simulink model "ForwardKinematic_YuMi"  (R2024a)
(part 22 of 23)

(4503599440548691*sin(q4R))/4503599627370496)*((7514214926474921*sin(q3R)*((4774755754024928798560446539205*cos(q2R))/10141204801825835211973625643008 + (7514214926474921*cos(q2R)*((3148506117433717*cos(q1R))/4503599627370496 + (1211728953682539*sin(q1R))/2251799813685248))/36893488147419103232 - sin(q2R)*((1211728953682539*cos(q1R))/2251799813685248 - (3148506117433717*sin(q1R))/4503599627370496)))/36893488147419103232 - cos(q3R)*((4774755754024928798560446539205*sin(q2R))/10141204801825835211973625643008 + cos(q2R)*((1211728953682539*cos(q1R))/2251799813685248 - (3148506117433717*sin(q1R))/4503599627370496) + (7514214926474921*sin(q2R)*((3148506117433717*cos(q1R))/4503599627370496 + (1211728953682539*sin(q1R))/2251799813685248))/36893488147419103232) + (9007199067919185*sin(q3R)*((28359221366286827792295350160645*cos(q1R))/40564819207303340847894502572032 + (10914283902180054573281797610715*sin(q1R))/20282409603651670423947251286016 - 3983318308679801924058395430653/41538374868278621028243970633760768))/9007199254740992) - ((9007199067919185*cos(q4R))/9007199254740992 - (234819211581865*sin(q4R))/1152921504606846976)*((213097284493758984364555654519459856780913684045*cos(q1R))/1496577676626844588240573268701473812127674924007424 - (43007175577195104036898489188735438973874147925*cos(q2R))/91343852333181432387730302044767688728495783936 + (82012275009546312639155898108543355135168378515*sin(q1R))/748288838313422294120286634350736906063837462003712 - (67682029681889335677290557259385*cos(q2R)*((3148506117433717*cos(q1R))/4503599627370496 + (1211728953682539*sin(q1R))/2251799813685248))/332306998946228968225951765070086144 + (9007199067919185*sin(q2R)*((1211728953682539*cos(q1R))/2251799813685248 - (3148506117433717*sin(q1R))/4503599627370496))/9007199254740992 - 29931509891982604486959633650198707742999153413/1532495540865888858358347027150309183618739122183602176) + (7514214926474921*sin(q4R)*((7514214926474921*cos(q3R)*((4774755754024928798560446539205*cos(q2R))/10141204801825835211973625643008 + (7514214926474921*cos(q2R)*((3148506117433717*cos(q1R))/4503599627370496 + (1211728953682539*sin(q1R))/2251799813685248))/36893488147419103232 - sin(q2R)*((1211728953682539*cos(q1R))/2251799813685248 - (3148506117433717*sin(q1R))/4503599627370496)))/36893488147419103232 + sin(q3R)*((4774755754024928798560446539205*sin(q2R))/10141204801825835211973625643008 + cos(q2R)*((1211728953682539*cos(q1R))/2251799813685248 - (3148506117433717*sin(q1R))/4503599627370496) + (7514214926474921*sin(q2R)*((3148506117433717*cos(q1R))/4503599627370496 + (1211728953682539*sin(q1R))/2251799813685248))/36893488147419103232) + (9007199067919185*cos(q3R)*((28359221366286827792295350160645*cos(q1R))/40564819207303340847894502572032 + (10914283902180054573281797610715*sin(q1R))/20282409603651670423947251286016 - 3983318308679801924058395430653/41538374868278621028243970633760768))/9007199254740992))/36893488147419103232))/36893488147419103232 + cos(q5R)*(((4503599440548691*cos(q4R))/4503599627370496 - (7514214926474921*sin(q4R))/36893488147419103232)*((7514214926474921*sin(q3R)*((4774755754024928798560446539205*cos(q2R))/10141204801825835211973625643008 + (7514214926474921*cos(q2R)*((3148506117433717*cos(q1R))/4503599627370496 + (1211728953682539*sin(q1R))/2251799813685248))/36893488147419103232 - sin(q2R)*((1211728953682539*cos(q1R))/2251799813685248 - (3148506117433717*sin(q1R))/4503599627370496)))/36893488147419103232 - cos(q3R)*((4774755754024928798560446539205*sin(q2R))/10141204801825835211973625643008 + cos(q2R)*((1211728953682539*cos(q1R))/2251799813685248 - (3148506117433717*sin(q1R))/4503599627370496) + (7514214926474921*sin(q2R)*((3148506117433717*cos(q1R))/4503599627370496 + (1211728953682539*sin(q1R))/2251799813685248))/36893488147419103232) + (9007199067919185*sin(q3R)*((28359221366286827792295350160645*cos(q1R))/40564819207303340847894502572032 + (10914283902180054573281797610715*sin(q1R))/20282409603651670423947251286016 - 3983318308679801924058395430653/41538374868278621028243970633760768))/9007199254740992) + ((234819211581865*cos(q4R))/1152921504606846976 + (9007199067919185*sin(q4R))/9007199254740992)*((213097284493758984364555654519459856780913684045*cos(q1R))/1496577676626844588240573268701473812127674924007424 - (43007175577195104036898489188735438973874147925*cos(q2R))/91343852333181432387730302044767688728495783936 + (82012275009546312639155898108543355135168378515*sin(q1R))/748288838313422294120286634350736906063837462003712 - (67682029681889335677290557259385*cos(q2R)*((3148506117433717*cos(q1R))/4503599627370496 + (1211728953682539*sin(q1R))/2251799813685248))/332306998946228968225951765070086144 + (9007199067919185*sin(q2R)*((1211728953682539*cos(q1R))/2251799813685248 - (3148506117433717*sin(q1R))/4503599627370496))/9007199254740992 - 29931509891982604486959633650198707742999153413/1532495540865888858358347027150309183618739122183602176) + (7514214926474921*cos(q4R)*((7514214926474921*cos(q3R)*((4774755754024928798560446539205*cos(q2R))/10141204801825835211973625643008 + (7514214926474921*cos(q2R)*((3148506117433717*cos(q1R))/4503599627370496 + (1211728953682539*sin(q1R))/2251799813685248))/36893488147419103232 - sin(q2R)*((1211728953682539*cos(q1R))/2251799813685248 - (3148506117433717*sin(q1R))/4503599627370496)))/36893488147419103232 + sin(q3R)*((4774755754024928798560446539205*sin(q2R))/10141204801825835211973625643008 + cos(q2R)*((1211728953682539*cos(q1R))/2251799813685248 - (3148506117433717*sin(q1R))/4503599627370496) + (7514214926474921*sin(q2R)*((3148506117433717*cos(q1R))/4503599627370496 + (1211728953682539*sin(q1R))/2251799813685248))/36893488147419103232) + (9007199067919185*cos(q3R)*((28359221366286827792295350160645*cos(q1R))/40564819207303340847894502572032 + (10914283902180054573281797610715*sin(q1R))/20282409603651670423947251286016 - 3983318308679801924058395430653/41538374868278621028243970633760768))/9007199254740992))/36893488147419103232)))/9007199254740992000 + (81*((4503599440548691*cos(q4R))/4503599627370496 - (7514214926474921*sin(q4R))/36893488147419103232)*((7514214926474921*sin(q3R)*((4774755754024928798560446539205*cos(q2R))/10141204801825835211973625643008 + (7514214926474921*cos(q2R)*((3148506117433717*cos(q1R))/4503599627370496 + (1211728953682539*sin(q1R))/2251799813685248))/36893488147419103232 - sin(q2R)*((1211728953682539*cos(q1R))/2251799813685248 - (3148506117433717*sin(q1R))/4503599627370496)))/36893488147419103232 - cos(q3R)*((4774755754024928798560446539205*sin(q2R))/10141204801825835211973625643008 + cos(q2R)*((1211728953682539*cos(q1R))/2251799813685248 - (3148506117433717*sin(q1R))/4503599627370496) + (7514214926474921*sin(q2R)*((3148506117433717*cos(q1R))/4503599627370496 + (1211728953682539*sin(q1R))/2251799813685248))/36893488147419103232) + (9007199067919185*sin(q3R)*((28359221366286827792295350160645*cos(q1R))/40564819207303340847894502572032 + (10914283902180054573281797610715*sin(q1R))/20282409603651670423947251286016 - 3983318308679801924058395430653/41538374868278621028243970633760768))/9007199254740992))/2000 - (81222263116692158804177042061221826384594597321566869716687*((7514214926474921*cos(q4R))/36893488147419103232 + (4503599440548691*sin(q4R))/4503599627370496)*((7514214926474921*sin(q3R)*((4774755754024928798560446539205*cos(q2R))/10141204801825835211973625643008 + (7514214926474921*cos(q2R)*((3148506117433717*cos(q1R))/4503599627370496 + (1211728953682539*sin(q1R))/2251799813685248))/36893488147419103232 - sin(q2R)*((1211728953682539*cos(q1R))/2251799813685248 - (3148506117433717*sin(q1R))/4503599627370496)))/36893488147419103232 - cos(q3R)*((4774755754024928798560446539205*sin(q2R))/10141204801825835211973625643008 + cos(q2R)*((1211728953682539*cos(q1R))/2251799813685248 - (3148506117433717*sin(q1R))/4503599627370496) + (7514214926474921*sin(q2R)*((3148506117433717*cos(q1R))/4503599627370496 + (1211728953682539*sin(q1R))/2251799813685248))/36893488147419103232) + (9007199067919185*sin(q3R)*((28359221366286827792295350160645*cos(q1R))/40564819207303340847894502572032 + (10914283902180054573281797610715*sin(q1R))/20282409603651670423947251286016 - 3983318308679801924058395430653/41538374868278621028243970633760768))/9007199254740992))/306499108173177771671669405430061836723747824436720435200000 + (81222263116692158804177042061221826384594597321566869716687*((9007199067919185*cos(q4R))/9007199254740992 - (234819211581865*sin(q4R))/1152921504606846976)*((213097284493758984364555654519459856780913684045*cos(q1R))/1496577676626844588240573268701473812127674924007424 - (43007175577195104036898489188735438973874147925*cos(q2R))/91343852333181432387730302044767688728495783936 + (82012275009546312639155898108543355135168378515*sin(q1R))/748288838313422294120286634350736906063837462003712 - (67682029681889335677290557259385*cos(q2R)*((3148506117433717*cos(q1R))/4503599627370496 + (1211728953682539*sin(q1R))/2251799813685248))/332306998946228968225951765070086144 + (9007199067919185*sin(q2R)*((1211728953682539*cos(q1R))/2251799813685248 - (3148506117433717*sin(q1R))/4503599627370496))/9007199254740992 - 29931509891982604486959633650198707742999153413/1532495540865888858358347027150309183618739122183602176))/306499108173177771671669405430061836723747824436720435200000 + (81*((234819211581865*cos(q4R))/1152921504606846976 + (9007199067919185*sin(q4R))/9007199254740992)*((213097284493758984364555654519459856780913684045*cos(q1R))/1496577676626844588240573268701473812127674924007424 - (43007175577195104036898489188735438973874147925*cos(q2R))/91343852333181432387730302044767688728495783936 + (82012275009546312639155898108543355135168378515*sin(q1R))/748288838313422294120286634350736906063837462003712 - (67682029681889335677290557259385*cos(q2R)*((3148506117433717*cos(q1R))/4503599627370496 + (1211728953682539*sin(q1R))/2251799813685248))/332306998946228968225951765070086144 + (9007199067919185*sin(q2R)*((1211728953682539*cos(q1R))/2251799813685248 - (3148506117433717*sin(q1R))/4503599627370496))/9007199254740992 - 29931509891982604486959633650198707742999153413/1532495540865888858358347027150309183618739122183602176))/2000 - (584133382113593486367040631332731*cos(q6R)*((9007199067919185*((7514214926474921*cos(q4R))/36893488147419103232 + (4503599440548691*sin(q4R))/4503599627370496)*((7514214926474921*sin(q3R)*((4774755754024928798560446539205*cos(q2R))/10141204801825835211973625643008 + (7514214926474921*cos(q2R)*((3148506117433717*cos(q1R))/4503599627370496 + (1211728953682539*sin(q1R))/2251799813685248))/36893488147419103232 - sin(q2R)*((1211728953682539*cos(q1R))/2251799813685248 - (3148506117433717*sin(q1R))/4503599627370496)))/36893488147419103232 - cos(q3R)*((4774755754024928798560446539205*sin(q2R))/10141204801825835211973625643008 + cos(q2R)*((1211728953682539*cos(q1R))/2251799813685248 - (3148506117433717*sin(q1R))/4503599627370496) + (7514214926474921*sin(q2R)*((3148506117433717*cos(q1R))/4503599627370496 + (1211728953682539*sin(q1R))/2251799813685248))/36893488147419103232) + (9007199067919185*sin(q3R)*((28359221366286827792295350160645*cos(q1R))/40564819207303340847894502572032 + (10914283902180054573281797610715*sin(q1R))/20282409603651670423947251286016 - 3983318308679801924058395430653/41538374868278621028243970633760768))/9007199254740992))/9007199254740992 - (9007199067919185*((9007199067919185*cos(q4R))/9007199254740992 - (234819211581865*sin(q4R))/1152921504606846976)*((213097284493758984364555654519459856780913684045*cos(q1R))/1496577676626844588240573268701473812127674924007424 - (43007175577195104036898489188735438973874147925*cos(q2R))/91343852333181432387730302044767688728495783936 + (82012275009546312639155898108543355135168378515*sin(q1R))/748288838313422294120286634350736906063837462003712 - (67682029681889335677290557259385*cos(q2R)*((3148506117433717*cos(q1R))/4503599627370496 + (1211728953682539*sin(q1R))/2251799813685248))/332306998946228968225951765070086144 + (9007199067919185*sin(q2R)*((1211728953682539*cos(q1R))/2251799813685248 - (3148506117433717*sin(q1R))/4503599627370496))/9007199254740992 - 29931509891982604486959633650198707742999153413/1532495540865888858358347027150309183618739122183602176))/9007199254740992 + (67682029681889335677290557259385*sin(q4R)*((7514214926474921*cos(q3R)*((4774755754024928798560446539205*cos(q2R))/10141204801825835211973625643008 + (7514214926474921*cos(q2R)*((3148506117433717*cos(q1R))/4503599627370496 + (1211728953682539*sin(q1R))/2251799813685248))/36893488147419103232 - sin(q2R)*((1211728953682539*cos(q1R))/2251799813685248 - (3148506117433717*sin(q1R))/4503599627370496)))/36893488147419103232 + sin(q3R)*((4774755754024928798560446539205*sin(q2R))/10141204801825835211973625643008 + cos(q2R)*((1211728953682539*cos(q1R))/2251799813685248 - (3148506117433717*sin(q1R))/4503599627370496) + (7514214926474921*sin(q2R)*((3148506117433717*cos(q1R))/4503599627370496 + (1211728953682539*sin(q1R))/2251799813685248))/36893488147419103232) + (9007199067919185*cos(q3R)*((28359221366286827792295350160645*cos(q1R))/40564819207303340847894502572032 + (10914283902180054573281797610715*sin(q1R))/20282409603651670423947251286016 - 3983318308679801924058395430653/41538374868278621028243970633760768))/9007199254740992))/332306998946228968225951765070086144))/16225927682921336339157801028812800 - (48638874966763599*sin(q6R)*((9007199067919185*((7514214926474921*cos(q4R))/36893488147419103232 + (4503599440548691*sin(q4R))/4503599627370496)*((7514214926474921*sin(q3R)*((4774755754024928798560446539205*cos(q2R))/10141204801825835211973625643008 + (7514214926474921*cos(q2R)*((3148506117433717*cos(q1R))/4503599627370496 + (1211728953682539*sin(q1R))/2251799813685248))/36893488147419103232 - sin(q2R)*((1211728953682539*cos(q1R))/2251799813685248 - (3148506117433717*sin(q1R))/4503599627370496)))/36893488147419103232 - cos(q3R)*((4774755754024928798560446539205*sin(q2R))/10141204801825835211973625643008 + cos(q2R)*((1211728953682539*cos(q1R))/2251799813685248 - (3148506117433717*sin(q1R))/4503599627370496) + (7514214926474921*sin(q2R)*((3148506117433717*cos(q1R))/4503599627370496 + (1211728953682539*sin(q1R))/2251799813685248))/36893488147419103232) + (9007199067919185*sin(q3R)*((28359221366286827792295350160645*cos(q1R))/40564819207303340847894502572032 + (10914283902180054573281797610715*sin(q1R))/20282409603651670423947251286016 - 3983318308679801924058395430653/41538374868278621028243970633760768))/9007199254740992))/9007199254740992 - (9007199067919185*((9007199067919185*cos(q4R))/9007199254740992 - (234819211581865*sin(q4R))/1152921504606846976)*((213097284493758984364555654519459856780913684045*cos(q1R))/1496577676626844588240573268701473812127674924007424 - (43007175577195104036898489188735438973874147925*cos(q2R))/91343852333181432387730302044767688728495783936 + (82012275009546312639155898108543355135168378515*sin(q1R))/748288838313422294120286634350736906063837462003712 - (67682029681889335677290557259385*cos(q2R)*((3148506117433717*cos(q1R))/4503599627370496 + (1211728953682539*sin(q1R))/2251799813685248))/332306998946228968225951765070086144 + (9007199067919185*sin(q2R)*((1211728953682539*cos(q1R))/2251799813685248 - (3148506117433717*sin(q1R))/4503599627370496))/9007199254740992 - 29931509891982604486959633650198707742999153413/1532495540865888858358347027150309183618739122183602176))/9007199254740992 + (67682029681889335677290557259385*sin(q4R)*((7514214926474921*cos(q3R)*((4774755754024928798560446539205*cos(q2R))/10141204801825835211973625643008 + (7514214926474921*cos(q2R)*((3148506117433717*cos(q1R))/4503599627370496 + (1211728953682539*sin(q1R))/2251799813685248))/36893488147419103232 - sin(q2R)*((1211728953682539*cos(q1R))/2251799813685248 - (3148506117433717*sin(q1R))/4503599627370496)))/36893488147419103232 + sin(q3R)*((4774755754024928798560446539205*sin(q2R))/10141204801825835211973625643008 + cos(q2R)*((1211728953682539*cos(q1R))/2251799813685248 - (3148506117433717*sin(q1R))/4503599627370496) + (7514214926474921*sin(q2R)*((3148506117433717*cos(q1R))/4503599627370496 + (1211728953682539*sin(q1R))/2251799813685248))/36893488147419103232) + (9007199067919185*cos(q3R)*((28359221366286827792295350160645*cos(q1R))/40564819207303340847894502572032 + (10914283902180054573281797610715*sin(q1R))/20282409603651670423947251286016 - 3983318308679801924058395430653/41538374868278621028243970633760768))/9007199254740992))/332306998946228968225951765070086144))/1801439850948198400 + (608651409044468601*cos(q4R)*((7514214926474921*cos(q3R)*((4774755754024928798560446539205*cos(q2R))/10141204801825835211973625643008 + (7514214926474921*cos(q2R)*((3148506117433717*cos(q1R))/4503599627370496 + (1211728953682539*sin(q1R))/2251799813685248))/36893488147419103232 - sin(q2R)*((1211728953682539*cos(q1R))/2251799813685248 - (3148506117433717*sin(q1R))/4503599627370496)))/36893488147419103232 + sin(q3R)*((4774755754024928798560446539205*sin(q2R))/10141204801825835211973625643008 + cos(q2R)*((1211728953682539*cos(q1R))/2251799813685248 - (3148506117433717*sin(q1R))/4503599627370496) + (7514214926474921*sin(q2R)*((3148506117433717*cos(q1R))/4503599627370496 + (1211728953682539*sin(q1R))/2251799813685248))/36893488147419103232) + (9007199067919185*cos(q3R)*((28359221366286827792295350160645*cos(q1R))/40564819207303340847894502572032 + (10914283902180054573281797610715*sin(q1R))/20282409603651670423947251286016 - 3983318308679801924058395430653/41538374868278621028243970633760768))/9007199254740992))/73786976294838206464000 - (27*cos(q5R)*(((4503599440548691*cos(q4R))/4503599627370496 - (7514214926474921*sin(q4R))/36893488147419103232)*((7514214926474921*sin(q3R)*((4774755754024928798560446539205*cos(q2R))/10141204801825835211973625643008 + (7514214926474921*cos(q2R)*((3148506117433717*cos(q1R))/4503599627370496 + (1211728953682539*sin(q1R))/2251799813685248))/36893488147419103232 - sin(q2R)*((1211728953682539*cos(q1R))/2251799813685248 - (3148506117433717*sin(q1R))/4503599627370496)))/36893488147419103232 - cos(q3R)*((4774755754024928798560446539205*sin(q2R))/10141204801825835211973625643008 + cos(q2R)*((1211728953682539*cos(q1R))/2251799813685248 - (3148506117433717*sin(q1R))/4503599627370496) + (7514214926474921*sin(q2R)*((3148506117433717*cos(q1R))/4503599627370496 + (1211728953682539*sin(q1R))/2251799813685248))/36893488147419103232) + (9007199067919185*sin(q3R)*((28359221366286827792295350160645*cos(q1R))/40564819207303340847894502572032 + (10914283902180054573281797610715*sin(q1R))/20282409603651670423947251286016 - 3983318308679801924058395430653/41538374868278621028243970633760768))/9007199254740992) + ((234819211581865*cos(q4R))/1152921504606846976 + (9007199067919185*sin(q4R))/9007199254740992)*((213097284493758984364555654519459856780913684045*cos(q1R))/1496577676626844588240573268701473812127674924007424 - (43007175577195104036898489188735438973874147925*cos(q2R))/91343852333181432387730302044767688728495783936 + (82012275009546312639155898108543355135168378515*sin(q1R))/748288838313422294120286634350736906063837462003712 - (67682029681889335677290557259385*cos(q2R)*((3148506117433717*cos(q1R))/4503599627370496 + (1211728953682539*sin(q1R))/2251799813685248))/332306998946228968225951765070086144 + (9007199067919185*sin(q2R)*((1211728953682539*cos(q1R))/2251799813685248 - (3148506117433717*sin(q1R))/4503599627370496))/9007199254740992 - 29931509891982604486959633650198707742999153413/1532495540865888858358347027150309183618739122183602176) + (7514214926474921*cos(q4R)*((7514214926474921*cos(q3R)*((4774755754024928798560446539205*cos(q2R))/10141204801825835211973625643008 + (7514214926474921*cos(q2R)*((3148506117433717*cos(q1R))/4503599627370496 + (1211728953682539*sin(q1R))/2251799813685248))/36893488147419103232 - sin(q2R)*((1211728953682539*cos(q1R))/2251799813685248 - (3148506117433717*sin(q1R))/4503599627370496)))/36893488147419103232 + sin(q3R)*((4774755754024928798560446539205*sin(q2R))/10141204801825835211973625643008 + cos(q2R)*((1211728953682539*cos(q1R))/2251799813685248 - (3148506117433717*sin(q1R))/4503599627370496) + (7514214926474921*sin(q2R)*((3148506117433717*cos(q1R))/4503599627370496 + (1211728953682539*sin(q1R))/2251799813685248))/36893488147419103232) + (9007199067919185*cos(q3R)*((28359221366286827792295350160645*cos(q1R))/40564819207303340847894502572032 + (10914283902180054573281797610715*sin(q1R))/20282409603651670423947251286016 - 3983318308679801924058395430653/41538374868278621028243970633760768))/9007199254740992))/36893488147419103232))/1000 - (610321541873521657855151997354401418608858870661075444886782706002880706727*sin(q4R)*((7514214926474921*cos(q3R)*((4774755754024928798560446539205*cos(q2R))/10141204801825835211973625643008 + (7514214926474921*cos(q2R)*((3148506117433717*cos(q1R))/4503599627370496 + (1211728953682539*sin(q1R))/2251799813685248))/36893488147419103232 - sin(q2R)*((1211728953682539*cos(q1R))/2251799813685248 - (3148506117433717*sin(q1R))/4503599627370496)))/36893488147419103232 + sin(q3R)*((4774755754024928798560446539205*sin(q2R))/10141204801825835211973625643008 + cos(q2R)*((1211728953682539*cos(q1R))/2251799813685248 - (3148506117433717*sin(q1R))/4503599627370496) + (7514214926474921*sin(q2R)*((3148506117433717*cos(q1R))/4503599627370496 + (1211728953682539*sin(q1R))/2251799813685248))/36893488147419103232) + (9007199067919185*cos(q3R)*((28359221366286827792295350160645*cos(q1R))/40564819207303340847894502572032 + (10914283902180054573281797610715*sin(q1R))/20282409603651670423947251286016 - 3983318308679801924058395430653/41538374868278621028243970633760768))/9007199254740992))/11307821214581659709333104004754678501295896940003961331978279688272766566400000 - (94754841554645069948206780163139*sin(q5R)*(((4503599440548691*cos(q4R))/4503599627370496 - (7514214926474921*sin(q4R))/36893488147419103232)*((7514214926474921*sin(q3R)*((4774755754024928798560446539205*cos(q2R))/10141204801825835211973625643008 + (7514214926474921*cos(q2R)*((3148506117433717*cos(q1R))/4503599627370496 + (1211728953682539*sin(q1R))/2251799813685248))/36893488147419103232 - sin(q2R)*((1211728953682539*cos(q1R))/2251799813685248 - (3148506117433717*sin(q1R))/4503599627370496)))/36893488147419103232 - cos(q3R)*((4774755754024928798560446539205*sin(q2R))/10141204801825835211973625643008 + cos(q2R)*((1211728953682539*cos(q1R))/2251799813685248 - (3148506117433717*sin(q1R))/4503599627370496) + (7514214926474921*sin(q2R)*((3148506117433717*cos(q1R))/4503599627370496 + (1211728953682539*sin(q1R))/2251799813685248))/36893488147419103232) + (9007199067919185*sin(q3R)*((28359221366286827792295350160645*cos(q1R))/40564819207303340847894502572032 + (10914283902180054573281797610715*sin(q1R))/20282409603651670423947251286016 - 3983318308679801924058395430653/41538374868278621028243970633760768))/9007199254740992) + ((234819211581865*cos(q4R))/1152921504606846976 + (9007199067919185*sin(q4R))/9007199254740992)*((213097284493758984364555654519459856780913684045*cos(q1R))/1496577676626844588240573268701473812127674924007424 - (43007175577195104036898489188735438973874147925*cos(q2R))/91343852333181432387730302044767688728495783936 + (82012275009546312639155898108543355135168378515*sin(q1R))/748288838313422294120286634350736906063837462003712 - (67682029681889335677290557259385*cos(q2R)*((3148506117433717*cos(q1R))/4503599627370496 + (1211728953682539*sin(q1R))/2251799813685248))/332306998946228968225951765070086144 + (9007199067919185*sin(q2R)*((1211728953682539*cos(q1R))/2251799813685248 - (3148506117433717*sin(q1R))/4503599627370496))/9007199254740992 - 29931509891982604486959633650198707742999153413/1532495540865888858358347027150309183618739122183602176) + (7514214926474921*cos(q4R)*((7514214926474921*cos(q3R)*((4774755754024928798560446539205*cos(q2R))/10141204801825835211973625643008 + (7514214926474921*cos(q2R)*((3148506117433717*cos(q1R))/4503599627370496 + (1211728953682539*sin(q1R))/2251799813685248))/36893488147419103232 - sin(q2R)*((1211728953682539*cos(q1R))/2251799813685248 - (3148506117433717*sin(q1R))/4503599627370496)))/36893488147419103232 + sin(q3R)*((4774755754024928798560446539205*sin(q2R))/10141204801825835211973625643008 + cos(q2R)*((1211728953682539*cos(q1R))/2251799813685248 - (3148506117433717*sin(q1R))/4503599627370496) + (7514214926474921*sin(q2R)*((3148506117433717*cos(q1R))/4503599627370496 + (1211728953682539*sin(q1R))/2251799813685248))/36893488147419103232) + (9007199067919185*cos(q3R)*((28359221366286827792295350160645*cos(q1R))/40564819207303340847894502572032 + (10914283902180054573281797610715*sin(q1R))/20282409603651670423947251286016 - 3983318308679801924058395430653/41538374868278621028243970633760768))/9007199254740992))/36893488147419103232))/66461399789245793645190353014017228800 + (712008244765680093343103025701132101054572137019*cos(q5R)*(((7514214926474921*cos(q4R))/36893488147419103232 + (4503599440548691*sin(q4R))/4503599627370496)*((7514214926474921*sin(q3R)*((4774755754024928798560446539205*cos(q2R))/10141204801825835211973625643008 + (7514214926474921*cos(q2R)*((3148506117433717*cos(q1R))/4503599627370496 + (1211728953682539*sin(q1R))/2251799813685248))/36893488147419103232 - sin(q2R)*((1211728953682539*cos(q1R))/2251799813685248 - (3148506117433717*sin(q1R))/4503599627370496)))/36893488147419103232 - cos(q3R)*((4774755754024928798560446539205*sin(q2R))/10141204801825835211973625643008 + cos(q2R)*((1211728953682539*cos(q1R))/2251799813685248 - (3148506117433717*sin(q1R))/4503599627370496) + (7514214926474921*sin(q2R)*((3148506117433717*cos(q1R))/4503599627370496 + (1211728953682539*sin(q1R))/2251799813685248))/36893488147419103232) + (9007199067919185*sin(q3R)*((28359221366286827792295350160645*cos(q1R))/40564819207303340847894502572032 + (10914283902180054573281797610715*sin(q1R))/20282409603651670423947251286016 - 3983318308679801924058395430653/41538374868278621028243970633760768))/9007199254740992) - ((9007199067919185*cos(q4R))/9007199254740992 - (234819211581865*sin(q4R))/1152921504606846976)*((213097284493758984364555654519459856780913684045*cos(q1R))/1496577676626844588240573268701473812127674924007424 - (43007175577195104036898489188735438973874147925*cos(q2R))/91343852333181432387730302044767688728495783936 + (82012275009546312639155898108543355135168378515*sin(q1R))/748288838313422294120286634350736906063837462003712 - (67682029681889335677290557259385*cos(q2R)*((3148506117433717*cos(q1R))/4503599627370496 + (1211728953682539*sin(q1R))/2251799813685248))/332306998946228968225951765070086144 + (9007199067919185*sin(q2R)*((1211728953682539*cos(q1R))/2251799813685248 - (3148506117433717*sin(q1R))/4503599627370496))/9007199254740992 - 29931509891982604486959633650198707742999153413/1532495540865888858358347027150309183618739122183602176) + (7514214926474921*sin(q4R)*((7514214926474921*cos(q3R)*((4774755754024928798560446539205*cos(q2R))/10141204801825835211973625643008 + (7514214926474921*cos(q2R)*((3148506117433717*cos(q1R))/4503599627370496 + (1211728953682539*sin(q1R))/2251799813685248))/36893488147419103232 - sin(q2R)*((1211728953682539*cos(q1R))/2251799813685248 - (3148506117433717*sin(q1R))/4503599627370496)))/36893488147419103232 + sin(q3R)*((4774755754024928798560446539205*sin(q2R))/10141204801825835211973625643008 + cos(q2R)*((1211728953682539*cos(q1R))/2251799813685248 - (3148506117433717*sin(q1R))/4503599627370496) + (7514214926474921*sin(q2R)*((3148506117433717*cos(q1R))/4503599627370496 + (1211728953682539*sin(q1R))/2251799813685248))/36893488147419103232) + (9007199067919185*cos(q3R)*((28359221366286827792295350160645*cos(q1R))/40564819207303340847894502572032 + (10914283902180054573281797610715*sin(q1R))/20282409603651670423947251286016 - 3983318308679801924058395430653/41538374868278621028243970633760768))/9007199254740992))/36893488147419103232))/2451992865385422173373355243440494693789982595493763481600 + (2436553109258773196144549622003023*cos(q6R)*(sin(q5R)*(((4503599440548691*cos(q4R))/4503599627370496 - (7514214926474921*sin(q4R))/36893488147419103232)*((7514214926474921*sin(q3R)*((4774755754024928798560446539205*cos(q2R))/10141204801825835211973625643008 + (7514214926474921*cos(q2R)*((3148506117433717*cos(q1R))/4503599627370496 + (1211728953682539*sin(q1R))/2251799813685248))/36893488147419103232 - sin(q2R)*((1211728953682539*cos(q1R))/2251799813685248 - (3148506117433717*sin(q1R))/4503599627370496)))/36893488147419103232 - cos(q3R)*((4774755754024928798560446539205*sin(q2R))/10141204801825835211973625643008 + cos(q2R)*((1211728953682539*cos(q1R))/2251799813685248 - (3148506117433717*sin(q1R))/4503599627370496) + (7514214926474921*sin(q2R)*((3148506117433717*cos(q1R))/4503599627370496 + (1211728953682539*sin(q1R))/2251799813685248))/36893488147419103232) + (9007199067919185*sin(q3R)*((28359221366286827792295350160645*cos(q1R))/40564819207303340847894502572032 + (10914283902180054573281797610715*sin(q1R))/20282409603651670423947251286016 - 3983318308679801924058395430653/41538374868278621028243970633760768))/9007199254740992) + ((234819211581865*cos(q4R))/1152921504606846976 + (9007199067919185*sin(q4R))/9007199254740992)*((213097284493758984364555654519459856780913684045*cos(q1R))/1496577676626844588240573268701473812127674924007424 - (43007175577195104036898489188735438973874147925*cos(q2R))/91343852333181432387730302044767688728495783936 + (82012275009546312639155898108543355135168378515*sin(q1R))/748288838313422294120286634350736906063837462003712 - (67682029681889335677290557259385*cos(q2R)*((3148506117433717*cos(q1R))/4503599627370496 + (1211728953682539*sin(q1R))/2251799813685248))/332306998946228968225951765070086144 + (9007199067919185*sin(q2R)*((1211728953682539*cos(q1R))/2251799813685248 - (3148506117433717*sin(q1R))/4503599627370496))/9007199254740992 - 29931509891982604486959633650198707742999153413/1532495540865888858358347027150309183618739122183602176) + (7514214926474921*cos(q4R)*((7514214926474921*cos(q3R)*((4774755754024928798560446539205*cos(q2R))/10141204801825835211973625643008 + (7514214926474921*cos(q2R)*((3148506117433717*cos(q1R))/4503599627370496 + (1211728953682539*sin(q1R))/2251799813685248))/36893488147419103232 - sin(q2R)*((1211728953682539*cos(q1R))/2251799813685248 - (3148506117433717*sin(q1R))/4503599627370496)))/36893488147419103232 + sin(q3R)*((4774755754024928798560446539205*sin(q2R))/10141204801825835211973625643008 + cos(q2R)*((1211728953682539*cos(q1R))/2251799813685248 - (3148506117433717*sin(q1R))/4503599627370496) + (7514214926474921*sin(q2R)*((3148506117433717*cos(q1R))/4503599627370496 + (1211728953682539*sin(q1R))/2251799813685248))/36893488147419103232) + (9007199067919185*cos(q3R)*((28359221366286827792295350160645*cos(q1R))/40564819207303340847894502572032 + (10914283902180054573281797610715*sin(q1R))/20282409603651670423947251286016 - 3983318308679801924058395430653/41538374868278621028243970633760768))/9007199254740992))/36893488147419103232) - (7514214926474921*cos(q5R)*(((7514214926474921*cos(q4R))/36893488147419103232 + (4503599440548691*sin(q4R))/4503599627370496)*((7514214926474921*sin(q3R)*((4774755754024928798560446539205*cos(q2R))/10141204801825835211973625643008 + (7514214926474921*cos(q2R)*((3148506117433717*cos(q1R))/4503599627370496 + (1211728953682539*sin(q1R))/2251799813685248))/36893488147419103232 - sin(q2R)*((1211728953682539*cos(q1R))/2251799813685248 - (3148506117433717*sin(q1R))/4503599627370496)))/36893488147419103232 - cos(q3R)*((4774755754024928798560446539205*sin(q2R))/10141204801825835211973625643008 + cos(q2R)*((1211728953682539*cos(q1R))/2251799813685248 - (3148506117433717*sin(q1R))/4503599627370496) + (7514214926474921*sin(q2R)*((3148506117433717*cos(q1R))/4503599627370496 + (1211728953682539*sin(q1R))/2251799813685248))/36893488147419103232) + (9007199067919185*sin(q3R)*((28359221366286827792295350160645*cos(q1R))/40564819207303340847894502572032 + (10914283902180054573281797610715*sin(q1R))/20282409603651670423947251286016 - 3983318308679801924058395430653/41538374868278621028243970633760768))/9007199254740992) - ((9007199067919185*cos(q4R))/9007199254740992 - (234819211581865*sin(q4R))/1152921504606846976)*((213097284493758984364555654519459856780913684045*cos(q1R))/1496577676626844588240573268701473812127674924007424 - (43007175577195104036898489188735438973874147925*cos(q2R))/91343852333181432387730302044767688728495783936 + (82012275009546312639155898108543355135168378515*sin(q1R))/748288838313422294120286634350736906063837462003712 - (67682029681889335677290557259385*cos(q2R)*((3148506117433717*cos(q1R))/4503599627370496 + (1211728953682539*sin(q1R))/2251799813685248))/332306998946228968225951765070086144 + (9007199067919185*sin(q2R)*((1211728953682539*cos(q1R))/2251799813685248 - (3148506117433717*sin(q1R))/4503599627370496))/9007199254740992 - 29931509891982604486959633650198707742999153413/1532495540865888858358347027150309183618739122183602176) + (7514214926474921*sin(q4R)*((7514214926474921*cos(q3R)*((4774755754024928798560446539205*cos(q2R))/10141204801825835211973625643008 + (7514214926474921*cos(q2R)*((3148506117433717*cos(q1R))/4503599627370496 + (1211728953682539*sin(q1R))/2251799813685248))/36893488147419103232 - sin(q2R)*((1211728953682539*cos(q1R))/2251799813685248 - (3148506117433717*sin(q1R))/4503599627370496)))/36893488147419103232 + sin(q3R)*((4774755754024928798560446539205*sin(q2R))/10141204801825835211973625643008 + cos(q2R)*((1211728953682539*cos(q1R))/2251799813685248 - (3148506117433717*sin(q1R))/4503599627370496) + (7514214926474921*sin(q2R)*((3148506117433717*cos(q1R))/4503599627370496 + (1211728953682539*sin(q1R))/2251799813685248))/36893488147419103232) + (9007199067919185*cos(q3R)*((28359221366286827792295350160645*cos(q1R))/40564819207303340847894502572032 + (10914283902180054573281797610715*sin(q1R))/20282409603651670423947251286016 - 3983318308679801924058395430653/41538374868278621028243970633760768))/9007199254740992))/36893488147419103232))/36893488147419103232))/332306998946228968225951765070086144000 + (27*cos(q6R)*((7514214926474921*sin(q5R)*(((7514214926474921*cos(q4R))/36893488147419103232 + (4503599440548691*sin(q4R))/4503599627370496)*((7514214926474921*sin(q3R)*((4774755754024928798560446539205*cos(q2R))/10141204801825835211973625643008 + (7514214926474921*cos(q2R)*((3148506117433717*cos(q1R))/4503599627370496 + (1211728953682539*sin(q1R))/2251799813685248))/36893488147419103232 - sin(q2R)*((1211728953682539*cos(q1R))/2251799813685248 - (3148506117433717*sin(q1R))/4503599627370496)))/36893488147419103232 - cos(q3R)*((4774755754024928798560446539205*sin(q2R))/10141204801825835211973625643008 + cos(q2R)*((1211728953682539*cos(q1R))/2251799813685248 - (3148506117433717*sin(q1R))/4503599627370496) + (7514214926474921*sin(q2R)*((3148506117433717*cos(q1R))/4503599627370496 + (1211728953682539*sin(q1R))/2251799813685248))/36893488147419103232) + (9007199067919185*sin(q3R)*((28359221366286827792295350160645*cos(q1R))/40564819207303340847894502572032 + (10914283902180054573281797610715*sin(q1R))/20282409603651670423947251286016 - 3983318308679801924058395430653/41538374868278621028243970633760768))/9007199254740992) - ((9007199067919185*cos(q4R))/9007199254740992 - (234819211581865*sin(q4R))/1152921504606846976)*((213097284493758984364555654519459856780913684045*cos(q1R))/1496577676626844588240573268701473812127674924007424 - (43007175577195104036898489188735438973874147925*cos(q2R))/91343852333181432387730302044767688728495783936 + (82012275009546312639155898108543355135168378515*sin(q1R))/748288838313422294120286634350736906063837462003712 - (67682029681889335677290557259385*cos(q2R)*((3148506117433717*cos(q1R))/4503599627370496 + (1211728953682539*sin(q1R))/2251799813685248))/332306998946228968225951765070086144 + (9007199067919185*sin(q2R)*((1211728953682539*cos(q1R))/2251799813685248 - (3148506117433717*sin(q1R))/4503599627370496))/9007199254740992 - 29931509891982604486959633650198707742999153413/1532495540865888858358347027150309183618739122183602176) + (7514214926474921*sin(q4R)*((7514214926474921*cos(q3R)*((4774755754024928798560446539205*cos(q2R))/10141204801825835211973625643008 + (7514214926474921*cos(q2R)*((3148506117433717*cos(q1R))/4503599627370496 + (1211728953682539*sin(q1R))/2251799813685248))/36893488147419103232 - sin(q2R)*((1211728953682539*cos(q1R))/2251799813685248 - (3148506117433717*sin(q1R))/4503599627370496)))/36893488147419103232 + sin(q3R)*((4774755754024928798560446539205*sin(q2R))/10141204801825835211973625643008 + cos(q2R)*((1211728953682539*cos(q1R))/2251799813685248 - (3148506117433717*sin(q1R))/4503599627370496) + (7514214926474921*sin(q2R)*((3148506117433717*cos(q1R))/4503599627370496 + (1211728953682539*sin(q1R))/2251799813685248))/36893488147419103232) + (9007199067919185*cos(q3R)*((28359221366286827792295350160645*cos(q1R))/40564819207303340847894502572032 + (10914283902180054573281797610715*sin(q1R))/20282409603651670423947251286016 - 3983318308679801924058395430653/41538374868278621028243970633760768))/9007199254740992))/36893488147419103232))/36893488147419103232 + cos(q5R)*(((4503599440548691*cos(q4R))/4503599627370496 - (7514214926474921*sin(q4R))/36893488147419103232)*((7514214926474921*sin(q3R)*((4774755754024928798560446539205*cos(q2R))/10141204801825835211973625643008 + (7514214926474921*cos(q2R)*((3148506117433717*cos(q1R))/4503599627370496 + (1211728953682539*sin(q1R))/2251799813685248))/36893488147419103232 - sin(q2R)*((1211728953682539*cos(q1R))/2251799813685248 - (3148506117433717*sin(q1R))/4503599627370496)))/36893488147419103232 - cos(q3R)*((4774755754024928798560446539205*sin(q2R))/10141204801825835211973625643008 + cos(q2R)*((1211728953682539*cos(q1R))/2251799813685248 - (3148506117433717*sin(q1R))/4503599627370496) + (7514214926474921*sin(q2R)*((3148506117433717*cos(q1R))/4503599627370496 + (1211728953682539*sin(q1R))/2251799813685248))/36893488147419103232) + (9007199067919185*sin(q3R)*((28359221366286827792295350160645*cos(q1R))/40564819207303340847894502572032 + (10914283902180054573281797610715*sin(q1R))/20282409603651670423947251286016 - 3983318308679801924058395430653/41538374868278621028243970633760768))/9007199254740992) + ((234819211581865*cos(q4R))/1152921504606846976 + (9007199067919185*sin(q4R))/9007199254740992)*((213097284493758984364555654519459856780913684045*cos(q1R))/1496577676626844588240573268701473812127674924007424 - (43007175577195104036898489188735438973874147925*cos(q2R))/91343852333181432387730302044767688728495783936 + (82012275009546312639155898108543355135168378515*sin(q1R))/748288838313422294120286634350736906063837462003712 - (67682029681889335677290557259385*cos(q2R)*((3148506117433717*cos(q1R))/4503599627370496 + (1211728953682539*sin(q1R))/2251799813685248))/332306998946228968225951765070086144 + (9007199067919185*sin(q2R)*((1211728953682539*cos(q1R))/2251799813685248 - (3148506117433717*sin(q1R))/4503599627370496))/9007199254740992 - 29931509891982604486959633650198707742999153413/1532495540865888858358347027150309183618739122183602176) + (7514214926474921*cos(q4R)*((7514214926474921*cos(q3R)*((4774755754024928798560446539205*cos(q2R))/10141204801825835211973625643008 + (7514214926474921*cos(q2R)*((3148506117433717*cos(q1R))/4503599627370496 + (1211728953682539*sin(q1R))/2251799813685248))/36893488147419103232 - sin(q2R)*((1211728953682539*cos(q1R))/2251799813685248 - (3148506117433717*sin(q1R))/4503599627370496)))/36893488147419103232 + sin(q3R)*((4774755754024928798560446539205*sin(q2R))/10141204801825835211973625643008 + cos(q2R)*((1211728953682539*cos(q1R))/2251799813685248 - (3148506117433717*sin(q1R))/4503599627370496) + (7514214926474921*sin(q2R)*((3148506117433717*cos(q1R))/4503599627370496 + (1211728953682539*sin(q1R))/2251799813685248))/36893488147419103232) + (9007199067919185*cos(q3R)*((28359221366286827792295350160645*cos(q1R))/40564819207303340847894502572032 + (10914283902180054573281797610715*sin(q1R))/20282409603651670423947251286016 - 3983318308679801924058395430653/41538374868278621028243970633760768))/9007199254740992))/36893488147419103232)))/1000, (27*sin(q5R)*(((7514214926474921*cos(q4R))/36893488147419103232 + (4503599440548691*sin(q4R))/4503599627370496)*((7514214926474921*sin(q3R)*((4774755754024928798560446539205*cos(q2R))/10141204801825835211973625643008 + (7514214926474921*cos(q2R)*((3148506117433717*cos(q1R))/4503599627370496 + (1211728953682539*sin(q1R))/2251799813685248))/36893488147419103232 - sin(q2R)*((1211728953682539*cos(q1R))/2251799813685248 - (3148506117433717*sin(q1R))/4503599627370496)))/36893488147419103232 - cos(q3R)*((4774755754024928798560446539205*sin(q2R))/10141204801825835211973625643008 + cos(q2R)*((1211728953682539*cos(q1R))/2251799813685248 - (3148506117433717*sin(q1R))/4503599627370496) + (7514214926474921*sin(q2R)*((3148506117433717*cos(q1R))/4503599627370496 + (1211728953682539*sin(q1R))/2251799813685248))/36893488147419103232) + (9007199067919185*sin(q3R)*((28359221366286827792295350160645*cos(q1R))/40564819207303340847894502572032 + (10914283902180054573281797610715*sin(q1R))/20282409603651670423947251286016 - 3983318308679801924058395430653/41538374868278621028243970633760768))/9007199254740992) - ((9007199067919185*cos(q4R))/9007199254740992 - (234819211581865*sin(q4R))/1152921504606846976)*((213097284493758984364555654519459856780913684045*cos(q1R))/1496577676626844588240573268701473812127674924007424 - (43007175577195104036898489188735438973874147925*cos(q2R))/91343852333181432387730302044767688728495783936 + (82012275009546312639155898108543355135168378515*sin(q1R))/748288838313422294120286634350736906063837462003712 - (67682029681889335677290557259385*cos(q2R)*((3148506117433717*cos(q1R))/4503599627370496 + (1211728953682539*sin(q1R))/2251799813685248))/332306998946228968225951765070086144 + (9007199067919185*sin(q2R)*((1211728953682539*cos(q1R))/2251799813685248 - (3148506117433717*sin(q1R))/4503599627370496))/9007199254740992 - 29931509891982604486959633650198707742999153413/1532495540865888858358347027150309183618739122183602176) + (7514214926474921*sin(q4R)*((7514214926474921*cos(q3R)*((4774755754024928798560446539205*cos(q2R))/10141204801825835211973625643008 + (7514214926474921*cos(q2R)*((3148506117433717*cos(q1R))/4503599627370496 + (1211728953682539*sin(q1R))/2251799813685248))/36893488147419103232 - sin(q2R)*((1211728953682539*cos(q1R))/2251799813685248 - (3148506117433717*sin(q1R))/4503599627370496)))/36893488147419103232 + sin(q3R)*((4774755754024928798560446539205*sin(q2R))/10141204801825835211973625643008 + cos(q2R)*((1211728953682539*cos(q1R))/2251799813685248 - (3148506117433717*sin(q1R))/4503599627370496) + (7514214926474921*sin(q2R)*((3148506117433717*cos(q1R))/4503599627370496 + (1211728953682539*sin(q1R))/2251799813685248))/36893488147419103232) + (9007199067919185*cos(q3R)*((28359221366286827792295350160645*cos(q1R))/40564819207303340847894502572032 + (10914283902180054573281797610715*sin(q1R))/20282409603651670423947251286016 - 3983318308679801924058395430653/41538374868278621028243970633760768))/9007199254740992))/36893488147419103232))/1000 + (324259171862923063*sin(q6R)*(sin(q5R)*(((7514214926474921*cos(q4R))/36893488147419103232 + (4503599440548691*sin(q4R))/4503599627370496)*((7514214926474921*sin(q3R)*((4774755754024928798560446539205*cos(q2R))/10141204801825835211973625643008 + (7514214926474921*cos(q2R)*((3148506117433717*cos(q1R))/4503599627370496 + (1211728953682539*sin(q1R))/2251799813685248))/36893488147419103232 - sin(q2R)*((1211728953682539*cos(q1R))/2251799813685248 - (3148506117433717*sin(q1R))/4503599627370496)))/36893488147419103232 - cos(q3R)*((4774755754024928798560446539205*sin(q2R))/10141204801825835211973625643008 + cos(q2R)*((1211728953682539*cos(q1R))/2251799813685248 - (3148506117433717*sin(q1R))/4503599627370496) + (7514214926474921*sin(q2R)*((3148506117433717*cos(q1R))/4503599627370496 + (1211728953682539*sin(q1R))/2251799813685248))/36893488147419103232) + (9007199067919185*sin(q3R)*((28359221366286827792295350160645*cos(q1R))/40564819207303340847894502572032 + (10914283902180054573281797610715*sin(q1R))/20282409603651670423947251286016 - 3983318308679801924058395430653/41538374868278621028243970633760768))/9007199254740992) - ((9007199067919185*cos(q4R))/9007199254740992 - (234819211581865*sin(q4R))/1152921504606846976)*((213097284493758984364555654519459856780913684045*cos(q1R))/1496577676626844588240573268701473812127674924007424 - (43007175577195104036898489188735438973874147925*cos(q2R))/91343852333181432387730302044767688728495783936 + (82012275009546312639155898108543355135168378515*sin(q1R))/748288838313422294120286634350736906063837462003712 - (67682029681889335677290557259385*cos(q2R)*((3148506117433717*cos(q1R))/4503599627370496 + (1211728953682539*sin(q1R))/2251799813685248))/332306998946228968225951765070086144 + (9007199067919185*sin(q2R)*((1211728953682539*cos(q1R))/2251799813685248 - (3148506117433717*sin(q1R))/4503599627370496))/9007199254740992 - 29931509891982604486959633650198707742999153413/1532495540865888858358347027150309183618739122183602176) + (7514214926474921*sin(q4R)*((7514214926474921*cos(q3R)*((4774755754024928798560446539205*cos(q2R))/10141204801825835211973625643008 + (7514214926474921*cos(q2R)*((3148506117433717*cos(q1R))/4503599627370496 + (1211728953682539*sin(q1R))/2251799813685248))/36893488147419103232 - sin(q2R)*((1211728953682539*cos(q1R))/2251799813685248 - (3148506117433717*sin(q1R))/4503599627370496)))/36893488147419103232 + sin(q3R)*((4774755754024928798560446539205*sin(q2R))/10141204801825835211973625643008 + cos(q2R)*((1211728953682539*cos(q1R))/2251799813685248 - (3148506117433717*sin(q1R))/4503599627370496) + (7514214926474921*sin(q2R)*((3148506117433717*cos(q1R))/4503599627370496 + (1211728953682539*sin(q1R))/2251799813685248))/36893488147419103232) + (9007199067919185*cos(q3R)*((28359221366286827792295350160645*cos(q1R))/40564819207303340847894502572032 + (10914283902180054573281797610715*sin(q1R))/20282409603651670423947251286016 - 3983318308679801924058395430653/41538374868278621028243970633760768))/9007199254740992))/36893488147419103232) + (9007199067919185*cos(q5R)*((67399765602155231606998903473897443684277400996768941497011875*cos(q2R))/3450873173395281893717377931138512726225554486085193277581262111899648 - (333960713126929533372903469589741180908441336378844163830032875*cos(q1R))/56539106072908298546665520023773392506479484700019806659891398441363832832 - (128527577967104929471702655059245076724477257328642562920515125*sin(q1R))/28269553036454149273332760011886696253239742350009903329945699220681916416 + (106069577339469832923929692356850887620017617375*cos(q2R)*((3148506117433717*cos(q1R))/4503599627370496 + (1211728953682539*sin(q1R))/2251799813685248))/12554203470773361527671578846415332832204710888928069025792 + (67682029681889335677290557259385*cos(q3R)*((4774755754024928798560446539205*cos(q2R))/10141204801825835211973625643008 + (7514214926474921*cos(q2R)*((3148506117433717*cos(q1R))/4503599627370496 + (1211728953682539*sin(q1R))/2251799813685248))/36893488147419103232 - sin(q2R)*((1211728953682539*cos(q1R))/2251799813685248 - (3148506117433717*sin(q1R))/4503599627370496)))/332306998946228968225951765070086144 - (14115856197532180673579726082375*sin(q2R)*((1211728953682539*cos(q1R))/2251799813685248 - (3148506117433717*sin(q1R))/4503599627370496))/340282366920938463463374607431768211456 + (234819211581865*cos(q3R)*((4774755754024928798560446539205*sin(q2R))/10141204801825835211973625643008 + cos(q2R)*((1211728953682539*cos(q1R))/2251799813685248 - (3148506117433717*sin(q1R))/4503599627370496) + (7514214926474921*sin(q2R)*((3148506117433717*cos(q1R))/4503599627370496 + (1211728953682539*sin(q1R))/2251799813685248))/36893488147419103232))/1152921504606846976 - (1764482024691522628700660907665*sin(q3R)*((4774755754024928798560446539205*cos(q2R))/10141204801825835211973625643008 + (7514214926474921*cos(q2R)*((3148506117433717*cos(q1R))/4503599627370496 + (1211728953682539*sin(q1R))/2251799813685248))/36893488147419103232 - sin(q2R)*((1211728953682539*cos(q1R))/2251799813685248 - (3148506117433717*sin(q1R))/4503599627370496)))/42535295865117307932921825928971026432 + (9007199067919185*sin(q3R)*((4774755754024928798560446539205*sin(q2R))/10141204801825835211973625643008 + cos(q2R)*((1211728953682539*cos(q1R))/2251799813685248 - (3148506117433717*sin(q1R))/4503599627370496) + (7514214926474921*sin(q2R)*((3148506117433717*cos(q1R))/4503599627370496 + (1211728953682539*sin(q1R))/2251799813685248))/36893488147419103232))/9007199254740992 + (81129635049124235038645691064225*cos(q3R)*((28359221366286827792295350160645*cos(q1R))/40564819207303340847894502572032 + (10914283902180054573281797610715*sin(q1R))/20282409603651670423947251286016 - 3983318308679801924058395430653/41538374868278621028243970633760768))/81129638414606681695789005144064 - (2115063383689692319117831580025*sin(q3R)*((28359221366286827792295350160645*cos(q1R))/40564819207303340847894502572032 + (10914283902180054573281797610715*sin(q1R))/20282409603651670423947251286016 - 3983318308679801924058395430653/41538374868278621028243970633760768))/10384593717069655257060992658440192 + 46907910686140203564236702804319721336174201386222453025052275/57896044618658097711785492504343953926634992332820282019728792003956564819968))/9007199254740992 + (7514214926474921*cos(q5R)*(((4503599440548691*cos(q4R))/4503599627370496 - (7514214926474921*sin(q4R))/36893488147419103232)*((7514214926474921*sin(q3R)*((4774755754024928798560446539205*cos(q2R))/10141204801825835211973625643008 + (7514214926474921*cos(q2R)*((3148506117433717*cos(q1R))/4503599627370496 + (1211728953682539*sin(q1R))/2251799813685248))/36893488147419103232 - sin(q2R)*((1211728953682539*cos(q1R))/2251799813685248 - (3148506117433717*sin(q1R))/4503599627370496)))/36893488147419103232 - cos(q3R)*((4774755754024928798560446539205*sin(q2R))/10141204801825835211973625643008 + cos(q2R)*((1211728953682539*cos(q1R))/2251799813685248 - (3148506117433717*sin(q1R))/4503599627370496) + (7514214926474921*sin(q2R)*((3148506117433717*cos(q1R))/4503599627370496 + (1211728953682539*sin(q1R))/2251799813685248))/36893488147419103232) + (9007199067919185*sin(q3R)*((28359221366286827792295350160645*cos(q1R))/40564819207303340847894502572032 + (10914283902180054573281797610715*sin(q1R))/20282409603651670423947251286016 - 3983318308679801924058395430653/41538374868278621028243970633760768))/9007199254740992) + ((234819211581865*cos(q4R))/1152921504606846976 + (9007199067919185*sin(q4R))/9007199254740992)*((213097284493758984364555654519459856780913684045*cos(q1R))/1496577676626844588240573268701473812127674924007424 - (43007175577195104036898489188735438973874147925*cos(q2R))/91343852333181432387730302044767688728495783936 + (82012275009546312639155898108543355135168378515*sin(q1R))/748288838313422294120286634350736906063837462003712 - (67682029681889335677290557259385*cos(q2R)*((3148506117433717*cos(q1R))/4503599627370496 + (1211728953682539*sin(q1R))/2251799813685248))/332306998946228968225951765070086144 + (9007199067919185*sin(q2R)*((1211728953682539*cos(q1R))/2251799813685248 - (3148506117433717*sin(q1R))/4503599627370496))/9007199254740992 - 29931509891982604486959633650198707742999153413/1532495540865888858358347027150309183618739122183602176) + (7514214926474921*cos(q4R)*((7514214926474921*cos(q3R)*((4774755754024928798560446539205*cos(q2R))/10141204801825835211973625643008 + (7514214926474921*cos(q2R)*((3148506117433717*cos(q1R))/4503599627370496 + (1211728953682539*sin(q1R))/2251799813685248))/36893488147419103232 - sin(q2R)*((1211728953682539*cos(q1R))/2251799813685248 - (3148506117433717*sin(q1R))/4503599627370496)))/36893488147419103232 + sin(q3R)*((4774755754024928798560446539205*sin(q2R))/10141204801825835211973625643008 + cos(q2R)*((1211728953682539*cos(q1R))/2251799813685248 - (3148506117433717*sin(q1R))/4503599627370496) + (7514214926474921*sin(q2R)*((3148506117433717*cos(q1R))/4503599627370496 + (1211728953682539*sin(q1R))/2251799813685248))/36893488147419103232) + (9007199067919185*cos(q3R)*((28359221366286827792295350160645*cos(q1R))/40564819207303340847894502572032 + (10914283902180054573281797610715*sin(q1R))/20282409603651670423947251286016 - 3983318308679801924058395430653/41538374868278621028243970633760768))/9007199254740992))/36893488147419103232))/36893488147419103232))/9007199254740992000 - (2436553109258773196144549622003023*cos(q6R)*((9007199067919185*sin(q5R)*((67399765602155231606998903473897443684277400996768941497011875*cos(q2R))/3450873173395281893717377931138512726225554486085193277581262111899648 - (333960713126929533372903469589741180908441336378844163830032875*cos(q1R))/56539106072908298546665520023773392506479484700019806659891398441363832832 - (128527577967104929471702655059245076724477257328642562920515125*sin(q1R))/28269553036454149273332760011886696253239742350009903329945699220681916416 + (106069577339469832923929692356850887620017617375*cos(q2R)*((3148506117433717*cos(q1R))/4503599627370496 + (1211728953682539*sin(q1R))/2251799813685248))/12554203470773361527671578846415332832204710888928069025792 + (67682029681889335677290557259385*cos(q3R)*((4774755754024928798560446539205*cos(q2R))/10141204801825835211973625643008 + (7514214926474921*cos(q2R)*((3148506117433717*cos(q1R))/4503599627370496 + (1211728953682539*sin(q1R))/2251799813685248))/36893488147419103232 - sin(q2R)*((1211728953682539*cos(q1R))/2251799813685248 - (3148506117433717*sin(q1R))/4503599627370496)))/332306998946228968225951765070086144 - (14115856197532180673579726082375*sin(q2R)*((1211728953682539*cos(q1R))/2251799813685248 - (3148506117433717*sin(q1R))/4503599627370496))/340282366920938463463374607431768211456 + (234819211581865*cos(q3R)*((4774755754024928798560446539205*sin(q2R))/10141204801825835211973625643008 + cos(q2R)*((1211728953682539*cos(q1R))/2251799813685248 - (3148506117433717*sin(q1R))/4503599627370496) + (7514214926474921*sin(q2R)*((3148506117433717*cos(q1R))/4503599627370496 + (1211728953682539*sin(q1R))/2251799813685248))/36893488147419103232))/1152921504606846976 - (1764482024691522628700660907665*sin(q3R)*((4774755754024928798560446539205*cos(q2R))/10141204801825835211973625643008 + (7514214926474921*cos(q2R)*((3148506117433717*cos(q1R))/4503599627370496 + (1211728953682539*sin(q1R))/2251799813685248))/36893488147419103232 - sin(q2R)*((1211728953682539*cos(q1R))/2251799813685248 - (3148506117433717*sin(q1R))/4503599627370496)))/42535295865117307932921825928971026432 + (9007199067919185*sin(q3R)*((4774755754024928798560446539205*sin(q2R))/10141204801825835211973625643008 + cos(q2R)*((1211728953682539*cos(q1R))/2251799813685248 - (3148506117433717*sin(q1R))/4503599627370496) + (7514214926474921*sin(q2R)*((3148506117433717*cos(q1R))/4503599627370496 + (1211728953682539*sin(q1R))/2251799813685248))/36893488147419103232))/9007199254740992 + (81129635049124235038645691064225*cos(q3R)*((28359221366286827792295350160645*cos(q1R))/40564819207303340847894502572032 + (10914283902180054573281797610715*sin(q1R))/20282409603651670423947251286016 - 3983318308679801924058395430653/41538374868278621028243970633760768))/81129638414606681695789005144064 - (2115063383689692319117831580025*sin(q3R)*((28359221366286827792295350160645*cos(q1R))/40564819207303340847894502572032 + (10914283902180054573281797610715*sin(q1R))/20282409603651670423947251286016 - 3983318308679801924058395430653/41538374868278621028243970633760768))/10384593717069655257060992658440192 + 46907910686140203564236702804319721336174201386222453025052275/57896044618658097711785492504343953926634992332820282019728792003956564819968))/9007199254740992 + (7514214926474921*sin(q5R)*(((4503599440548691*cos(q4R))/4503599627370496 - (7514214926474921*sin(q4R))/36893488147419103232)*((7514214926474921*sin(q3R)*((4774755754024928798560446539205*cos(q2R))/10141204801825835211973625643008 + (7514214926474921*cos(q2R)*((3148506117433717*cos(q1R))/4503599627370496 + (1211728953682539*sin(q1R))/2251799813685248))/36893488147419103232 - sin(q2R)*((1211728953682539*cos(q1R))/2251799813685248 - (3148506117433717*sin(q1R))/4503599627370496)))/36893488147419103232 - cos(q3R)*((4774755754024928798560446539205*sin(q2R))/10141204801825835211973625643008 + cos(q2R)*((1211728953682539*cos(q1R))/2251799813685248 - (3148506117433717*sin(q1R))/4503599627370496) + (7514214926474921*sin(q2R)*((3148506117433717*cos(q1R))/4503599627370496 + (1211728953682539*sin(q1R))/2251799813685248))/36893488147419103232) + (9007199067919185*sin(q3R)*((28359221366286827792295350160645*cos(q1R))/40564819207303340847894502572032 + (10914283902180054573281797610715*sin(q1R))/20282409603651670423947251286016 - 3983318308679801924058395430653/41538374868278621028243970633760768))/9007199254740992) + ((234819211581865*cos(q4R))/1152921504606846976 + (9007199067919185*sin(q4R))/9007199254740992)*((213097284493758984364555654519459856780913684045*cos(q1R))/1496577676626844588240573268701473812127674924007424 - (43007175577195104036898489188735438973874147925*cos(q2R))/91343852333181432387730302044767688728495783936 + (82012275009546312639155898108543355135168378515*sin(q1R))/748288838313422294120286634350736906063837462003712 - (67682029681889335677290557259385*cos(q2R)*((3148506117433717*cos(q1R))/4503599627370496 + (1211728953682539*sin(q1R))/2251799813685248))/332306998946228968225951765070086144 + (9007199067919185*sin(q2R)*((1211728953682539*cos(q1R))/2251799813685248 - (3148506117433717*sin(q1R))/4503599627370496))/9007199254740992 - 29931509891982604486959633650198707742999153413/1532495540865888858358347027150309183618739122183602176) + (7514214926474921*cos(q4R)*((7514214926474921*cos(q3R)*((4774755754024928798560446539205*cos(q2R))/10141204801825835211973625643008 + (7514214926474921*cos(q2R)*((3148506117433717*cos(q1R))/4503599627370496 + (1211728953682539*sin(q1R))/2251799813685248))/36893488147419103232 - sin(q2R)*((1211728953682539*cos(q1R))/2251799813685248 - (3148506117433717*sin(q1R))/4503599627370496)))/36893488147419103232 + sin(q3R)*((4774755754024928798560446539205*sin(q2R))/10141204801825835211973625643008 + cos(q2R)*((1211728953682539*cos(q1R))/2251799813685248 - (3148506117433717*sin(q1R))/4503599627370496) + (7514214926474921*sin(q2R)*((3148506117433717*cos(q1R))/4503599627370496 + (1211728953682539*sin(q1R))/2251799813685248))/36893488147419103232) + (9007199067919185*cos(q3R)*((28359221366286827792295350160645*cos(q1R))/40564819207303340847894502572032 + (10914283902180054573281797610715*sin(q1R))/20282409603651670423947251286016 - 3983318308679801924058395430653/41538374868278621028243970633760768))/9007199254740992))/36893488147419103232))/36893488147419103232 - cos(q5R)*(((7514214926474921*cos(q4R))/36893488147419103232 + (4503599440548691*sin(q4R))/4503599627370496)*((7514214926474921*sin(q3R)*((4774755754024928798560446539205*cos(q2R))/10141204801825835211973625643008 + (7514214926474921*cos(q2R)*((3148506117433717*cos(q1R))/4503599627370496 + (1211728953682539*sin(q1R))/2251799813685248))/36893488147419103232 - sin(q2R)*((1211728953682539*cos(q1R))/2251799813685248 - (3148506117433717*sin(q1R))/4503599627370496)))/36893488147419103232 - cos(q3R)*((4774755754024928798560446539205*sin(q2R))/10141204801825835211973625643008 + cos(q2R)*((1211728953682539*cos(q1R))/2251799813685248 - (3148506117433717*sin(q1R))/4503599627370496) + (7514214926474921*sin(q2R)*((3148506117433717*cos(q1R))/4503599627370496 + (1211728953682539*sin(q1R))/2251799813685248))/36893488147419103232) + (9007199067919185*sin(q3R)*((28359221366286827792295350160645*cos(q1R))/40564819207303340847894502572032 + (10914283902180054573281797610715*sin(q1R))/20282409603651670423947251286016 - 3983318308679801924058395430653/41538374868278621028243970633760768))/9007199254740992) - ((9007199067919185*cos(q4R))/9007199254740992 - (234819211581865*sin(q4R))/1152921504606846976)*((213097284493758984364555654519459856780913684045*cos(q1R))/1496577676626844588240573268701473812127674924007424 - (43007175577195104036898489188735438973874147925*cos(q2R))/91343852333181432387730302044767688728495783936 + (82012275009546312639155898108543355135168378515*sin(q1R))/748288838313422294120286634350736906063837462003712 - (67682029681889335677290557259385*cos(q2R)*((3148506117433717*cos(q1R))/4503599627370496 + (1211728953682539*sin(q1R))/2251799813685248))/332306998946228968225951765070086144 + (9007199067919185*sin(q2R)*((1211728953682539*cos(q1R))/2251799813685248 - (3148506117433717*sin(q1R))/4503599627370496))/9007199254740992 - 29931509891982604486959633650198707742999153413/1532495540865888858358347027150309183618739122183602176) + (7514214926474921*sin(q4R)*((7514214926474921*cos(q3R)*((4774755754024928798560446539205*cos(q2R))/10141204801825835211973625643008 + (7514214926474921*cos(q2R)*((3148506117433717*cos(q1R))/4503599627370496 + (1211728953682539*sin(q1R))/2251799813685248))/36893488147419103232 - sin(q2R)*((1211728953682539*cos(q1R))/2251799813685248 - (3148506117433717*sin(q1R))/4503599627370496)))/36893488147419103232 + sin(q3R)*((4774755754024928798560446539205*sin(q2R))/10141204801825835211973625643008 + cos(q2R)*((1211728953682539*cos(q1R))/2251799813685248 - (3148506117433717*sin(q1R))/4503599627370496) + (7514214926474921*sin(q2R)*((3148506117433717*cos(q1R))/4503599627370496 + (1211728953682539*sin(q1R))/2251799813685248))/36893488147419103232) + (9007199067919185*cos(q3R)*((28359221366286827792295350160645*cos(q1R))/40564819207303340847894502572032 + (10914283902180054573281797610715*sin(q1R))/20282409603651670423947251286016 - 3983318308679801924058395430653/41538374868278621028243970633760768))/9007199254740992))/36893488147419103232)))/332306998946228968225951765070086144000 + (48638874966763599*cos(q5R)*((67399765602155231606998903473897443684277400996768941497011875*cos(q2R))/3450873173395281893717377931138512726225554486085193277581262111899648 - (333960713126929533372903469589741180908441336378844163830032875*cos(q1R))/56539106072908298546665520023773392506479484700019806659891398441363832832 - (128527577967104929471702655059245076724477257328642562920515125*sin(q1R))/28269553036454149273332760011886696253239742350009903329945699220681916416 + (106069577339469832923929692356850887620017617375*cos(q2R)*((3148506117433717*cos(q1R))/4503599627370496 + (1211728953682539*sin(q1R))/2251799813685248))/12554203470773361527671578846415332832204710888928069025792 + (67682029681889335677290557259385*cos(q3R)*((4774755754024928798560446539205*cos(q2R))/10141204801825835211973625643008 + (7514214926474921*cos(q2R)*((3148506117433717*cos(q1R))/4503599627370496 + (1211728953682539*sin(q1R))/2251799813685248))/36893488147419103232 - sin(q2R)*((1211728953682539*cos(q1R))/2251799813685248 - (3148506117433717*sin(q1R))/4503599627370496)))/332306998946228968225951765070086144 - (14115856197532180673579726082375*sin(q2R)*((1211728953682539*cos(q1R))/2251799813685248 - (3148506117433717*sin(q1R))/4503599627370496))/340282366920938463463374607431768211456 + (234819211581865*cos(q3R)*((4774755754024928798560446539205*sin(q2R))/10141204801825835211973625643008 + cos(q2R)*((1211728953682539*cos(q1R))/2251799813685248 - (3148506117433717*sin(q1R))/4503599627370496) + (7514214926474921*sin(q2R)*((3148506117433717*cos(q1R))/4503599627370496 + (1211728953682539*sin(q1R))/2251799813685248))/36893488147419103232))/1152921504606846976 - (1764482024691522628700660907665*sin(q3R)*((4774755754024928798560446539205*cos(q2R))/10141204801825835211973625643008 + (7514214926474921*cos(q2R)*((3148506117433717*cos(q1R))/4503599627370496 + (1211728953682539*sin(q1R))/2251799813685248))/36893488147419103232 - sin(q2R)*((1211728953682539*cos(q1R))/2251799813685248 - (3148506117433717*sin(q1R))/4503599627370496)))/42535295865117307932921825928971026432 + (9007199067919185*sin(q3R)*((4774755754024928798560446539205*sin(q2R))/10141204801825835211973625643008 + cos(q2R)*((1211728953682539*cos(q1R))/2251799813685248 - (3148506117433717*sin(q1R))/4503599627370496) + (7514214926474921*sin(q2R)*((3148506117433717*cos(q1R))/4503599627370496 + (1211728953682539*sin(q1R))/2251799813685248))/36893488147419103232))/9007199254740992 + (81129635049124235038645691064225*cos(q3R)*((28359221366286827792295350160645*cos(q1R))/40564819207303340847894502572032 + (10914283902180054573281797610715*sin(q1R))/20282409603651670423947251286016 - 3983318308679801924058395430653/41538374868278621028243970633760768))/81129638414606681695789005144064 - (2115063383689692319117831580025*sin(q3R)*((28359221366286827792295350160645*cos(q1R))/40564819207303340847894502572032 + (10914283902180054573281797610715*sin(q1R))/20282409603651670423947251286016 - 3983318308679801924058395430653/41538374868278621028243970633760768))/10384593717069655257060992658440192 + 46907910686140203564236702804319721336174201386222453025052275/57896044618658097711785492504343953926634992332820282019728792003956564819968))/1801439850948198400 - (202883803014822867*sin(q6R)*((9007199067919185*sin(q5R)*((67399765602155231606998903473897443684277400996768941497011875*cos(q2R))/3450873173395281893717377931138512726225554486085193277581262111899648 - (333960713126929533372903469589741180908441336378844163830032875*cos(q1R))/56539106072908298546665520023773392506479484700019806659891398441363832832 - (128527577967104929471702655059245076724477257328642562920515125*sin(q1R))/28269553036454149273332760011886696253239742350009903329945699220681916416 + (106069577339469832923929692356850887620017617375*cos(q2R)*((3148506117433717*cos(q1R))/4503599627370496 + (1211728953682539*sin(q1R))/2251799813685248))/12554203470773361527671578846415332832204710888928069025792 + (67682029681889335677290557259385*cos(q3R)*((4774755754024928798560446539205*cos(q2R))/10141204801825835211973625643008 + (7514214926474921*cos(q2R)*((3148506117433717*cos(q1R))/4503599627370496 + (1211728953682539*sin(q1R))/2251799813685248))/36893488147419103232 - sin(q2R)*((1211728953682539*cos(q1R))/2251799813685248 - (3148506117433717*sin(q1R))/4503599627370496)))/332306998946228968225951765070086144 - (14115856197532180673579726082375*sin(q2R)*((1211728953682539*cos(q1R))/2251799813685248 - (3148506117433717*sin(q1R))/4503599627370496))/340282366920938463463374607431768211456 + (234819211581865*cos(q3R)*((4774755754024928798560446539205*sin(q2R))/10141204801825835211973625643008 + cos(q2R)*((1211728953682539*cos(q1R))/2251799813685248 - (3148506117433717*sin(q1R))/4503599627370496) + (7514214926474921*sin(q2R)*((3148506117433717*cos(q1R))/4503599627370496 + (1211728953682539*sin(q1R))/2251799813685248))/36893488147419103232))/1152921504606846976 - (1764482024691522628700660907665*sin(q3R)*((4774755754024928798560446539205*cos(q2R))/10141204801825835211973625643008 + (7514214926474921*cos(q2R)*((3148506117433717*cos(q1R))/4503599627370496 + (1211728953682539*sin(q1R))/2251799813685248))/36893488147419103232 - sin(q2R)*((1211728953682539*cos(q1R))/2251799813685248 - (3148506117433717*sin(q1R))/4503599627370496)))/42535295865117307932921825928971026432 + (9007199067919185*sin(q3R)*((4774755754024928798560446539205*sin(q2R))/10141204801825835211973625643008 + cos(q2R)*((1211728953682539*cos(q1R))/2251799813685248 - (3148506117433717*sin(q1R))/4503599627370496) + (7514214926474921*sin(q2R)*((3148506117433717*cos(q1R))/4503599627370496 + (1211728953682539*sin(q1R))/2251799813685248))/36893488147419103232))/9007199254740992 + (81129635049124235038645691064225*cos(q3R)*((28359221366286827792295350160645*cos(q1R))/40564819207303340847894502572032 + (10914283902180054573281797610715*sin(q1R))/20282409603651670423947251286016 - 3983318308679801924058395430653/41538374868278621028243970633760768))/81129638414606681695789005144064 - (2115063383689692319117831580025*sin(q3R)*((28359221366286827792295350160645*cos(q1R))/40564819207303340847894502572032 + (10914283902180054573281797610715*sin(q1R))/20282409603651670423947251286016 - 3983318308679801924058395430653/41538374868278621028243970633760768))/10384593717069655257060992658440192 + 46907910686140203564236702804319721336174201386222453025052275/57896044618658097711785492504343953926634992332820282019728792003956564819968))/9007199254740992 + (7514214926474921*sin(q5R)*(((4503599440548691*cos(q4R))/4503599627370496 - (7514214926474921*sin(q4R))/36893488147419103232)*((7514214926474921*sin(q3R)*((4774755754024928798560446539205*cos(q2R))/10141204801825835211973625643008 + (7514214926474921*cos(q2R)*((3148506117433717*cos(q1R))/4503599627370496 + (1211728953682539*sin(q1R))/2251799813685248))/36893488147419103232 - sin(q2R)*((1211728953682539*cos(q1R))/2251799813685248 - (3148506117433717*sin(q1R))/4503599627370496)))/36893488147419103232 - cos(q3R)*((4774755754024928798560446539205*sin(q2R))/10141204801825835211973625643008 + cos(q2R)*((1211728953682539*cos(q1R))/2251799813685248 - (3148506117433717*sin(q1R))/4503599627370496) + (7514214926474921*sin(q2R)*((3148506117433717*cos(q1R))/4503599627370496 + (1211728953682539*sin(q1R))/2251799813685248))/36893488147419103232) + (9007199067919185*sin(q3R)*((28359221366286827792295350160645*cos(q1R))/40564819207303340847894502572032 + (10914283902180054573281797610715*sin(q1R))/20282409603651670423947251286016 - 3983318308679801924058395430653/41538374868278621028243970633760768))/9007199254740992) + ((234819211581865*cos(q4R))/1152921504606846976 + (9007199067919185*sin(q4R))/9007199254740992)*((213097284493758984364555654519459856780913684045*cos(q1R))/1496577676626844588240573268701473812127674924007424 - (43007175577195104036898489188735438973874147925*cos(q2R))/91343852333181432387730302044767688728495783936 + (82012275009546312639155898108543355135168378515*sin(q1R))/748288838313422294120286634350736906063837462003712 - (67682029681889335677290557259385*cos(q2R)*((3148506117433717*cos(q1R))/4503599627370496 + (1211728953682539*sin(q1R))/2251799813685248))/332306998946228968225951765070086144 + (9007199067919185*sin(q2R)*((1211728953682539*cos(q1R))/2251799813685248 - (3148506117433717*sin(q1R))/4503599627370496))/9007199254740992 - 29931509891982604486959633650198707742999153413/1532495540865888858358347027150309183618739122183602176) + (7514214926474921*cos(q4R)*((7514214926474921*cos(q3R)*((4774755754024928798560446539205*cos(q2R))/10141204801825835211973625643008 + (7514214926474921*cos(q2R)*((3148506117433717*cos(q1R))/4503599627370496 + (1211728953682539*sin(q1R))/2251799813685248))/36893488147419103232 - sin(q2R)*((1211728953682539*cos(q1R))/2251799813685248 - (3148506117433717*sin(q1R))/4503599627370496)))/36893488147419103232 + sin(q3R)*((4774755754024928798560446539205*sin(q2R))/10141204801825835211973625643008 + cos(q2R)*((1211728953682539*cos(q1R))/2251799813685248 - (3148506117433717*sin(q1R))/4503599627370496) + (7514214926474921*sin(q2R)*((3148506117433717*cos(q1R))/4503599627370496 + (1211728953682539*sin(q1R))/2251799813685248))/36893488147419103232) + (9007199067919185*cos(q3R)*((28359221366286827792295350160645*cos(q1R))/40564819207303340847894502572032 + (10914283902180054573281797610715*sin(q1R))/20282409603651670423947251286016 - 3983318308679801924058395430653/41538374868278621028243970633760768))/9007199254740992))/36893488147419103232))/36893488147419103232 - cos(q5R)*(((7514214926474921*cos(q4R))/36893488147419103232 + (4503599440548691*sin(q4R))/4503599627370496)*((7514214926474921*sin(q3R)*((4774755754024928798560446539205*cos(q2R))/10141204801825835211973625643008 + (7514214926474921*cos(q2R)*((3148506117433717*cos(q1R))/4503599627370496 + (1211728953682539*sin(q1R))/2251799813685248))/36893488147419103232 - sin(q2R)*((1211728953682539*cos(q1R))/2251799813685248 - (3148506117433717*sin(q1R))/4503599627370496)))/36893488147419103232 - cos(q3R)*((4774755754024928798560446539205*sin(q2R))/10141204801825835211973625643008 + cos(q2R)*((1211728953682539*cos(q1R))/2251799813685248 - (3148506117433717*sin(q1R))/4503599627370496) + (7514214926474921*sin(q2R)*((3148506117433717*cos(q1R))/4503599627370496 + (1211728953682539*sin(q1R))/2251799813685248))/36893488147419103232) + (9007199067919185*sin(q3R)*((28359221366286827792295350160645*cos(q1R))/40564819207303340847894502572032 + (10914283902180054573281797610715*sin(q1R))/20282409603651670423947251286016 - 3983318308679801924058395430653/41538374868278621028243970633760768))/9007199254740992) - ((9007199067919185*cos(q4R))/9007199254740992 - (234819211581865*sin(q4R))/1152921504606846976)*((213097284493758984364555654519459856780913684045*cos(q1R))/1496577676626844588240573268701473812127674924007424 - (43007175577195104036898489188735438973874147925*cos(q2R))/91343852333181432387730302044767688728495783936 + (82012275009546312639155898108543355135168378515*sin(q1R))/748288838313422294120286634350736906063837462003712 - (67682029681889335677290557259385*cos(q2R)*((3148506117433717*cos(q1R))/4503599627370496 + (1211728953682539*sin(q1R))/2251799813685248))/332306998946228968225951765070086144 + (9007199067919185*sin(q2R)*((1211728953682539*cos(q1R))/2251799813685248 - (3148506117433717*sin(q1R))/4503599627370496))/9007199254740992 - 29931509891982604486959633650198707742999153413/1532495540865888858358347027150309183618739122183602176) + (7514214926474921*sin(q4R)*((7514214926474921*cos(q3R)*((4774755754024928798560446539205*cos(q2R))/10141204801825835211973625643008 + (7514214926474921*cos(q2R)*((3148506117433717*cos(q1R))/4503599627370496 + (1211728953682539*sin(q1R))/2251799813685248))/36893488147419103232 - sin(q2R)*((1211728953682539*cos(q1R))/2251799813685248 - (3148506117433717*sin(q1R))/4503599627370496)))/36893488147419103232 + sin(q3R)*((4774755754024928798560446539205*sin(q2R))/10141204801825835211973625643008 + cos(q2R)*((1211728953682539*cos(q1R))/2251799813685248 - (3148506117433717*sin(q1R))/4503599627370496) + (7514214926474921*sin(q2R)*((3148506117433717*cos(q1R))/4503599627370496 + (1211728953682539*sin(q1R))/2251799813685248))/36893488147419103232) + (9007199067919185*cos(q3R)*((28359221366286827792295350160645*cos(q1R))/40564819207303340847894502572032 + (10914283902180054573281797610715*sin(q1R))/20282409603651670423947251286016 - 3983318308679801924058395430653/41538374868278621028243970633760768))/9007199254740992))/36893488147419103232)))/36893488147419103232000 + (170695144106365826517608855445768431563113584343*sin(q5R)*((67399765602155231606998903473897443684277400996768941497011875*cos(q2R))/3450873173395281893717377931138512726225554486085193277581262111899648 - (333960713126929533372903469589741180908441336378844163830032875*cos(q1R))/56539106072908298546665520023773392506479484700019806659891398441363832832 - (128527577967104929471702655059245076724477257328642562920515125*sin(q1R))/28269553036454149273332760011886696253239742350009903329945699220681916416 + (106069577339469832923929692356850887620017617375*cos(q2R)*((3148506117433717*cos(q1R))/4503599627370496 + (1211728953682539*sin(q1R))/2251799813685248))/12554203470773361527671578846415332832204710888928069025792 + (67682029681889335677290557259385*cos(q3R)*((4774755754024928798560446539205*cos(q2R))/10141204801825835211973625643008 + (7514214926474921*cos(q2R)*((3148506117433717*cos(q1R))/4503599627370496 + (1211728953682539*sin(q1R))/2251799813685248))/36893488147419103232 - sin(q2R)*((1211728953682539*cos(q1R))/2251799813685248 - (3148506117433717*sin(q1R))/4503599627370496)))/332306998946228968225951765070086144 - (14115856197532180673579726082375*sin(q2R)*((1211728953682539*cos(q1R))/2251799813685248 - (3148506117433717*sin(q1R))/4503599627370496))/340282366920938463463374607431768211456 + (234819211581865*cos(q3R)*((4774755754024928798560446539205*sin(q2R))/10141204801825835211973625643008 + cos(q2R)*((1211728953682539*cos(q1R))/2251799813685248 - (3148506117433717*sin(q1R))/4503599627370496) + (7514214926474921*sin(q2R)*((3148506117433717*cos(q1R))/4503599627370496 + (1211728953682539*sin(q1R))/2251799813685248))/36893488147419103232))/1152921504606846976 - (1764482024691522628700660907665*sin(q3R)*((4774755754024928798560446539205*cos(q2R))/10141204801825835211973625643008 + (7514214926474921*cos(q2R)*((3148506117433717*cos(q1R))/4503599627370496 + (1211728953682539*sin(q1R))/2251799813685248))/36893488147419103232 - sin(q2R)*((1211728953682539*cos(q1R))/2251799813685248 - (3148506117433717*sin(q1R))/4503599627370496)))/42535295865117307932921825928971026432 + (9007199067919185*sin(q3R)*((4774755754024928798560446539205*sin(q2R))/10141204801825835211973625643008 + cos(q2R)*((1211728953682539*cos(q1R))/2251799813685248 - (3148506117433717*sin(q1R))/4503599627370496) + (7514214926474921*sin(q2R)*((3148506117433717*cos(q1R))/4503599627370496 + (1211728953682539*sin(q1R))/2251799813685248))/36893488147419103232))/9007199254740992 + (81129635049124235038645691064225*cos(q3R)*((28359221366286827792295350160645*cos(q1R))/40564819207303340847894502572032 + (10914283902180054573281797610715*sin(q1R))/20282409603651670423947251286016 - 3983318308679801924058395430653/41538374868278621028243970633760768))/81129638414606681695789005144064 - (2115063383689692319117831580025*sin(q3R)*((28359221366286827792295350160645*cos(q1R))/40564819207303340847894502572032 + (10914283902180054573281797610715*sin(q1R))/20282409603651670423947251286016 - 3983318308679801924058395430653/41538374868278621028243970633760768))/10384593717069655257060992658440192 + 46907910686140203564236702804319721336174201386222453025052275/57896044618658097711785492504343953926634992332820282019728792003956564819968))/119726214130147567059245861496117904970213993920593920 + (202883803014822867*cos(q5R)*(((4503599440548691*cos(q4R))/4503599627370496 - (7514214926474921*sin(q4R))/36893488147419103232)*((7514214926474921*sin(q3R)*((4774755754024928798560446539205*cos(q2R))/10141204801825835211973625643008 + (7514214926474921*cos(q2R)*((3148506117433717*cos(q1R))/4503599627370496 + (1211728953682539*sin(q1R))/2251799813685248))/36893488147419103232 - sin(q2R)*((1211728953682539*cos(q1R))/2251799813685248 - (3148506117433717*sin(q1R))/4503599627370496)))/36893488147419103232 - cos(q3R)*((4774755754024928798560446539205*sin(q2R))/10141204801825835211973625643008 + cos(q2R)*((1211728953682539*cos(q1R))/2251799813685248 - (3148506117433717*sin(q1R))/4503599627370496) + (7514214926474921*sin(q2R)*((3148506117433717*cos(q1R))/4503599627370496 + (1211728953682539*sin(q1R))/2251799813685248))/36893488147419103232) + (9007199067919185*sin(q3R)*((28359221366286827792295350160645*cos(q1R))/40564819207303340847894502572032 + (10914283902180054573281797610715*sin(q1R))/20282409603651670423947251286016 - 3983318308679801924058395430653/41538374868278621028243970633760768))/9007199254740992) + ((234819211581865*cos(q4R))/1152921504606846976 + (9007199067919185*sin(q4R))/9007199254740992)*((213097284493758984364555654519459856780913684045*cos(q1R))/1496577676626844588240573268701473812127674924007424 - (43007175577195104036898489188735438973874147925*cos(q2R))/91343852333181432387730302044767688728495783936 + (82012275009546312639155898108543355135168378515*sin(q1R))/748288838313422294120286634350736906063837462003712 - (67682029681889335677290557259385*cos(q2R)*((3148506117433717*cos(q1R))/4503599627370496 + (1211728953682539*sin(q1R))/2251799813685248))/332306998946228968225951765070086144 + (9007199067919185*sin(q2R)*((1211728953682539*cos(q1R))/2251799813685248 - (3148506117433717*sin(q1R))/4503599627370496))/9007199254740992 - 29931509891982604486959633650198707742999153413/1532495540865888858358347027150309183618739122183602176) + (7514214926474921*cos(q4R)*((7514214926474921*cos(q3R)*((4774755754024928798560446539205*cos(q2R))/10141204801825835211973625643008 + (7514214926474921*cos(q2R)*((3148506117433717*cos(q1R))/4503599627370496 + (1211728953682539*sin(q1R))/2251799813685248))/36893488147419103232 - sin(q2R)*((1211728953682539*cos(q1R))/2251799813685248 - (3148506117433717*sin(q1R))/4503599627370496)))/36893488147419103232 + sin(q3R)*((4774755754024928798560446539205*sin(q2R))/10141204801825835211973625643008 + cos(q2R)*((1211728953682539*cos(q1R))/2251799813685248 - (3148506117433717*sin(q1R))/4503599627370496) + (7514214926474921*sin(q2R)*((3148506117433717*cos(q1R))/4503599627370496 + (1211728953682539*sin(q1R))/2251799813685248))/36893488147419103232) + (9007199067919185*cos(q3R)*((28359221366286827792295350160645*cos(q1R))/40564819207303340847894502572032 + (10914283902180054573281797610715*sin(q1R))/20282409603651670423947251286016 - 3983318308679801924058395430653/41538374868278621028243970633760768))/9007199254740992))/36893488147419103232))/36893488147419103232000 + (712008244765680093343103025701132101054572137019*sin(q5R)*(((4503599440548691*cos(q4R))/4503599627370496 - (7514214926474921*sin(q4R))/36893488147419103232)*((7514214926474921*sin(q3R)*((4774755754024928798560446539205*cos(q2R))/10141204801825835211973625643008 + (7514214926474921*cos(q2R)*((3148506117433717*cos(q1R))/4503599627370496 + (1211728953682539*sin(q1R))/2251799813685248))/36893488147419103232 - sin(q2R)*((1211728953682539*cos(q1R))/2251799813685248 - (3148506117433717*sin(q1R))/4503599627370496)))/36893488147419103232 - cos(q3R)*((4774755754024928798560446539205*sin(q2R))/10141204801825835211973625643008 + cos(q2R)*((1211728953682539*cos(q1R))/2251799813685248 - (3148506117433717*sin(q1R))/4503599627370496) + (7514214926474921*sin(q2R)*((3148506117433717*cos(q1R))/4503599627370496 + (1211728953682539*sin(q1R))/2251799813685248))/36893488147419103232) + (9007199067919185*sin(q3R)*((28359221366286827792295350160645*cos(q1R))/40564819207303340847894502572032 + (10914283902180054573281797610715*sin(q1R))/20282409603651670423947251286016 - 3983318308679801924058395430653/41538374868278621028243970633760768))/9007199254740992) + ((234819211581865*cos(q4R))/1152921504606846976 + (9007199067919185*sin(q4R))/9007199254740992)*((213097284493758984364555654519459856780913684045*cos(q1R))/1496577676626844588240573268701473812127674924007424 - (43007175577195104036898489188735438973874147925*cos(q2R))/91343852333181432387730302044767688728495783936 + (82012275009546312639155898108543355135168378515*sin(q1R))/748288838313422294120286634350736906063837462003712 - (67682029681889335677290557259385*cos(q2R)*((3148506117433717*cos(q1R))/4503599627370496 + (1211728953682539*sin(q1R))/2251799813685248))/332306998946228968225951765070086144 + (9007199067919185*sin(q2R)*((1211728953682539*cos(q1R))/2251799813685248 - (3148506117433717*sin(q1R))/4503599627370496))/9007199254740992 - 29931509891982604486959633650198707742999153413/1532495540865888858358347027150309183618739122183602176) + (7514214926474921*cos(q4R)*((7514214926474921*cos(q3R)*((4774755754024928798560446539205*cos(q2R))/10141204801825835211973625643008 + (7514214926474921*cos(q2R)*((3148506117433717*cos(q1R))/4503599627370496 + (1211728953682539*sin(q1R))/2251799813685248))/36893488147419103232 - sin(q2R)*((1211728953682539*cos(q1R))/2251799813685248 - (3148506117433717*sin(q1R))/4503599627370496)))/36893488147419103232 + sin(q3R)*((4774755754024928798560446539205*sin(q2R))/10141204801825835211973625643008 + cos(q2R)*((1211728953682539*cos(q1R))/2251799813685248 - (3148506117433717*sin(q1R))/4503599627370496) + (7514214926474921*sin(q2R)*((3148506117433717*cos(q1R))/4503599627370496 + (1211728953682539*sin(q1R))/2251799813685248))/36893488147419103232) + (9007199067919185*cos(q3R)*((28359221366286827792295350160645*cos(q1R))/40564819207303340847894502572032 + (10914283902180054573281797610715*sin(q1R))/20282409603651670423947251286016 - 3983318308679801924058395430653/41538374868278621028243970633760768))/9007199254740992))/36893488147419103232))/2451992865385422173373355243440494693789982595493763481600 - (94754841554645069948206780163139*cos(q5R)*(((7514214926474921*cos(q4R))/36893488147419103232 + (4503599440548691*sin(q4R))/4503599627370496)*((7514214926474921*sin(q3R)*((4774755754024928798560446539205*cos(q2R))/10141204801825835211973625643008 + (7514214926474921*cos(q2R)*((3148506117433717*cos(q1R))/4503599627370496 + (1211728953682539*sin(q1R))/2251799813685248))/36893488147419103232 - sin(q2R)*((1211728953682539*cos(q1R))/2251799813685248 - (3148506117433717*sin(q1R))/4503599627370496)))/36893488147419103232 - cos(q3R)*((4774755754024928798560446539205*sin(q2R))/10141204801825835211973625643008 + cos(q2R)*((1211728953682539*cos(q1R))/2251799813685248 - (3148506117433717*sin(q1R))/4503599627370496) + (7514214926474921*sin(q2R)*((3148506117433717*cos(q1R))/4503599627370496 + (1211728953682539*sin(q1R))/2251799813685248))/36893488147419103232) + (9007199067919185*sin(q3R)*((28359221366286827792295350160645*cos(q1R))/40564819207303340847894502572032 + (10914283902180054573281797610715*sin(q1R))/20282409603651670423947251286016 - 3983318308679801924058395430653/41538374868278621028243970633760768))/9007199254740992) - ((9007199067919185*cos(q4R))/9007199254740992 - (234819211581865*sin(q4R))/1152921504606846976)*((213097284493758984364555654519459856780913684045*cos(q1R))/1496577676626844588240573268701473812127674924007424 - (43007175577195104036898489188735438973874147925*cos(q2R))/91343852333181432387730302044767688728495783936 + (82012275009546312639155898108543355135168378515*sin(q1R))/748288838313422294120286634350736906063837462003712 - (67682029681889335677290557259385*cos(q2R)*((3148506117433717*cos(q1R))/4503599627370496 + (1211728953682539*sin(q1R))/2251799813685248))/332306998946228968225951765070086144 + (9007199067919185*sin(q2R)*((1211728953682539*cos(q1R))/2251799813685248 - (3148506117433717*sin(q1R))/4503599627370496))/9007199254740992 - 29931509891982604486959633650198707742999153413/1532495540865888858358347027150309183618739122183602176) + (7514214926474921*sin(q4R)*((7514214926474921*cos(q3R)*((4774755754024928798560446539205*cos(q2R))/10141204801825835211973625643008 + (7514214926474921*cos(q2R)*((3148506117433717*cos(q1R))/4503599627370496 + (1211728953682539*sin(q1R))/2251799813685248))/36893488147419103232 - sin(q2R)*((1211728953682539*cos(q1R))/2251799813685248 - (3148506117433717*sin(q1R))/4503599627370496)))/36893488147419103232 + sin(q3R)*((4774755754024928798560446539205*sin(q2R))/10141204801825835211973625643008 + cos(q2R)*((1211728953682539*cos(q1R))/2251799813685248 - (3148506117433717*sin(q1R))/4503599627370496) + (7514214926474921*sin(q2R)*((3148506117433717*cos(q1R))/4503599627370496 + (1211728953682539*sin(q1R))/2251799813685248))/36893488147419103232) + (9007199067919185*cos(q3R)*((28359221366286827792295350160645*cos(q1R))/40564819207303340847894502572032 + (10914283902180054573281797610715*sin(q1R))/20282409603651670423947251286016 - 3983318308679801924058395430653/41538374868278621028243970633760768))/9007199254740992))/36893488147419103232))/66461399789245793645190353014017228800 - (27*cos(q6R)*(sin(q5R)*(((7514214926474921*cos(q4R))/36893488147419103232 + (4503599440548691*sin(q4R))/4503599627370496)*((7514214926474921*sin(q3R)*((4774755754024928798560446539205*cos(q2R))/10141204801825835211973625643008 + (7514214926474921*cos(q2R)*((3148506117433717*cos(q1R))/4503599627370496 + (1211728953682539*sin(q1R))/2251799813685248))/36893488147419103232 - sin(q2R)*((1211728953682539*cos(q1R))/2251799813685248 - (3148506117433717*sin(q1R))/4503599627370496)))/36893488147419103232 - cos(q3R)*((4774755754024928798560446539205*sin(q2R))/10141204801825835211973625643008 + cos(q2R)*((1211728953682539*cos(q1R))/2251799813685248 - (3148506117433717*sin(q1R))/4503599627370496) + (7514214926474921*sin(q2R)*((3148506117433717*cos(q1R))/4503599627370496 + (1211728953682539*sin(q1R))/2251799813685248))/36893488147419103232) + (9007199067919185*sin(q3R)*((28359221366286827792295350160645*cos(q1R))/40564819207303340847894502572032 + (10914283902180054573281797610715*sin(q1R))/20282409603651670423947251286016 - 3983318308679801924058395430653/41538374868278621028243970633760768))/9007199254740992) - ((9007199067919185*cos(q4R))/9007199254740992 - (234819211581865*sin(q4R))/1152921504606846976)*((213097284493758984364555654519459856780913684045*cos(q1R))/1496577676626844588240573268701473812127674924007424 - (43007175577195104036898489188735438973874147925*cos(q2R))/91343852333181432387730302044767688728495783936 + (82012275009546312639155898108543355135168378515*sin(q1R))/748288838313422294120286634350736906063837462003712 - (67682029681889335677290557259385*cos(q2R)*((3148506117433717*cos(q1R))/4503599627370496 + (1211728953682539*sin(q1R))/2251799813685248))/332306998946228968225951765070086144 + (9007199067919185*sin(q2R)*((1211728953682539*cos(q1R))/2251799813685248 - (3148506117433717*sin(q1R))/4503599627370496))/9007199254740992 - 29931509891982604486959633650198707742999153413/1532495540865888858358347027150309183618739122183602176) + (7514214926474921*sin(q4R)*((7514214926474921*cos(q3R)*((4774755754024928798560446539205*cos(q2R))/10141204801825835211973625643008 + (7514214926474921*cos(q2R)*((3148506117433717*cos(q1R))/4503599627370496 + (1211728953682539*sin(q1R))/2251799813685248))/36893488147419103232 - sin(q2R)*((1211728953682539*cos(q1R))/2251799813685248 - (3148506117433717*sin(q1R))/4503599627370496)))/36893488147419103232 + sin(q3R)*((4774755754024928798560446539205*sin(q2R))/10141204801825835211973625643008 + cos(q2R)*((1211728953682539*cos(q1R))/2251799813685248 - (3148506117433717*sin(q1R))/4503599627370496) + (7514214926474921*sin(q2R)*((3148506117433717*cos(q1R))/4503599627370496 + (1211728953682539*sin(q1R))/2251799813685248))/36893488147419103232) + (9007199067919185*cos(q3R)*((28359221366286827792295350160645*cos(q1R))/40564819207303340847894502572032 + (10914283902180054573281797610715*sin(q1R))/20282409603651670423947251286016 - 3983318308679801924058395430653/41538374868278621028243970633760768))/9007199254740992))/36893488147419103232) + (9007199067919185*cos(q5R)*((67399765602155231606998903473897443684277400996768941497011875*cos(q2R))/3450873173395281893717377931138512726225554486085193277581262111899648 - (333960713126929533372903469589741180908441336378844163830032875*cos(q1R))/56539106072908298546665520023773392506479484700019806659891398441363832832 - (128527577967104929471702655059245076724477257328642562920515125*sin(q1R))/28269553036454149273332760011886696253239742350009903329945699220681916416 + (106069577339469832923929692356850887620017617375*cos(q2R)*((3148506117433717*cos(q1R))/4503599627370496 + (1211728953682539*sin(q1R))/2251799813685248))/12554203470773361527671578846415332832204710888928069025792 + (67682029681889335677290557259385*cos(q3R)*((4774755754024928798560446539205*cos(q2R))/10141204801825835211973625643008 + (7514214926474921*cos(q2R)*((3148506117433717*cos(q1R))/4503599627370496 + (1211728953682539*sin(q1R))/2251799813685248))/36893488147419103232 - sin(q2R)*((1211728953682539*cos(q1R))/2251799813685248 - (3148506117433717*sin(q1R))/4503599627370496)))/332306998946228968225951765070086144 - (14115856197532180673579726082375*sin(q2R)*((1211728953682539*cos(q1R))/2251799813685248 - (3148506117433717*sin(q1R))/4503599627370496))/340282366920938463463374607431768211456 + (234819211581865*cos(q3R)*((4774755754024928798560446539205*sin(q2R))/10141204801825835211973625643008 + cos(q2R)*((1211728953682539*cos(q1R))/2251799813685248 - (3148506117433717*sin(q1R))/4503599627370496) + (7514214926474921*sin(q2R)*((3148506117433717*cos(q1R))/4503599627370496 + (1211728953682539*sin(q1R))/2251799813685248))/36893488147419103232))/1152921504606846976 - (1764482024691522628700660907665*sin(q3R)*((4774755754024928798560446539205*cos(q2R))/10141204801825835211973625643008 + (7514214926474921*cos(q2R)*((3148506117433717*cos(q1R))/4503599627370496 + (1211728953682539*sin(q1R))/2251799813685248))/36893488147419103232 - sin(q2R)*((1211728953682539*cos(q1R))/2251799813685248 - (3148506117433717*sin(q1R))/4503599627370496)))/42535295865117307932921825928971026432 + (9007199067919185*sin(q3R)*((4774755754024928798560446539205*sin(q2R))/10141204801825835211973625643008 + cos(q2R)*((1211728953682539*cos(q1R))/2251799813685248 - (3148506117433717*sin(q1R))/4503599627370496) + (7514214926474921*sin(q2R)*((3148506117433717*cos(q1R))/4503599627370496 + (1211728953682539*sin(q1R))/2251799813685248))/36893488147419103232))/9007199254740992 + (81129635049124235038645691064225*cos(q3R)*((28359221366286827792295350160645*cos(q1R))/40564819207303340847894502572032 + (10914283902180054573281797610715*sin(q1R))/20282409603651670423947251286016 - 3983318308679801924058395430653/41538374868278621028243970633760768))/81129638414606681695789005144064 - (2115063383689692319117831580025*sin(q3R)*((28359221366286827792295350160645*cos(q1R))/40564819207303340847894502572032 + (10914283902180054573281797610715*sin(q1R))/20282409603651670423947251286016 - 3983318308679801924058395430653/41538374868278621028243970633760768))/10384593717069655257060992658440192 + 46907910686140203564236702804319721336174201386222453025052275/57896044618658097711785492504343953926634992332820282019728792003956564819968))/9007199254740992 + (7514214926474921*cos(q5R)*(((4503599440548691*cos(q4R))/4503599627370496 - (7514214926474921*sin(q4R))/36893488147419103232)*((7514214926474921*sin(q3R)*((4774755754024928798560446539205*cos(q2R))/10141204801825835211973625643008 + (7514214926474921*cos(q2R)*((3148506117433717*cos(q1R))/4503599627370496 + (1211728953682539*sin(q1R))/2251799813685248))/36893488147419103232 - sin(q2R)*((1211728953682539*cos(q1R))/2251799813685248 - (3148506117433717*sin(q1R))/4503599627370496)))/36893488147419103232 - cos(q3R)*((4774755754024928798560446539205*sin(q2R))/10141204801825835211973625643008 + cos(q2R)*((1211728953682539*cos(q1R))/2251799813685248 - (3148506117433717*sin(q1R))/4503599627370496) + (7514214926474921*sin(q2R)*((3148506117433717*cos(q1R))/4503599627370496 + (1211728953682539*sin(q1R))/2251799813685248))/36893488147419103232) + (9007199067919185*sin(q3R)*((28359221366286827792295350160645*cos(q1R))/40564819207303340847894502572032 + (10914283902180054573281797610715*sin(q1R))/20282409603651670423947251286016 - 3983318308679801924058395430653/41538374868278621028243970633760768))/9007199254740992) + ((234819211581865*cos(q4R))/1152921504606846976 + (9007199067919185*sin(q4R))/9007199254740992)*((213097284493758984364555654519459856780913684045*cos(q1R))/1496577676626844588240573268701473812127674924007424 - (43007175577195104036898489188735438973874147925*cos(q2R))/91343852333181432387730302044767688728495783936 + (82012275009546312639155898108543355135168378515*sin(q1R))/748288838313422294120286634350736906063837462003712 - (67682029681889335677290557259385*cos(q2R)*((3148506117433717*cos(q1R))/4503599627370496 + (1211728953682539*sin(q1R))/2251799813685248))/332306998946228968225951765070086144 + (9007199067919185*sin(q2R)*((1211728953682539*cos(q1R))/2251799813685248 - (3148506117433717*sin(q1R))/4503599627370496))/9007199254740992 - 29931509891982604486959633650198707742999153413/1532495540865888858358347027150309183618739122183602176) + (7514214926474921*cos(q4R)*((7514214926474921*cos(q3R)*((4774755754024928798560446539205*cos(q2R))/10141204801825835211973625643008 + (7514214926474921*cos(q2R)*((3148506117433717*cos(q1R))/4503599627370496 + (1211728953682539*sin(q1R))/2251799813685248))/36893488147419103232 - sin(q2R)*((1211728953682539*cos(q1R))/2251799813685248 - (3148506117433717*sin(q1R))/4503599627370496)))/36893488147419103232 + sin(q3R)*((4774755754024928798560446539205*sin(q2R))/10141204801825835211973625643008 + cos(q2R)*((1211728953682539*cos(q1R))/2251799813685248 - (3148506117433717*sin(q1R))/4503599627370496) + (7514214926474921*sin(q2R)*((3148506117433717*cos(q1R))/4503599627370496 + (1211728953682539*sin(q1R))/2251799813685248))/36893488147419103232) + (9007199067919185*cos(q3R)*((28359221366286827792295350160645*cos(q1R))/40564819207303340847894502572032 + (10914283902180054573281797610715*sin(q1R))/20282409603651670423947251286016 - 3983318308679801924058395430653/41538374868278621028243970633760768))/9007199254740992))/36893488147419103232))/36893488147419103232))/1000, (324259171862923063*cos(q6R)*((9007199067919185*sin(q5R)*((67399765602155231606998903473897443684277400996768941497011875*cos(q2R))/3450873173395281893717377931138512726225554486085193277581262111899648 - (333960713126929533372903469589741180908441336378844163830032875*cos(q1R))/56539106072908298546665520023773392506479484700019806659891398441363832832 - (128527577967104929471702655059245076724477257328642562920515125*sin(q1R))/28269553036454149273332760011886696253239742350009903329945699220681916416 + (106069577339469832923929692356850887620017617375*cos(q2R)*((3148506117433717*cos(q1R))/4503599627370496 + (1211728953682539*sin(q1R))/2251799813685248))/12554203470773361527671578846415332832204710888928069025792 + (67682029681889335677290557259385*cos(q3R)*((4774755754024928798560446539205*cos(q2R))/10141204801825835211973625643008 + (7514214926474921*cos(q2R)*((3148506117433717*cos(q1R))/4503599627370496 + (1211728953682539*sin(q1R))/2251799813685248))/36893488147419103232 - sin(q2R)*((1211728953682539*cos(q1R))/2251799813685248 - (3148506117433717*sin(q1R))/4503599627370496)))/332306998946228968225951765070086144 - (14115856197532180673579726082375*sin(q2R)*((1211728953682539*cos(q1R))/2251799813685248 - (3148506117433717*sin(q1R))/4503599627370496))/340282366920938463463374607431768211456 + (234819211581865*cos(q3R)*((4774755754024928798560446539205*sin(q2R))/10141204801825835211973625643008 + cos(q2R)*((1211728953682539*cos(q1R))/2251799813685248 - (3148506117433717*sin(q1R))/4503599627370496) + (7514214926474921*sin(q2R)*((3148506117433717*cos(q1R))/4503599627370496 + (1211728953682539*sin(q1R))/2251799813685248))/36893488147419103232))/1152921504606846976 - (1764482024691522628700660907665*sin(q3R)*((4774755754024928798560446539205*cos(q2R))/10141204801825835211973625643008 + (7514214926474921*cos(q2R)*((3148506117433717*cos(q1R))/4503599627370496 + (1211728953682539*sin(q1R))/2251799813685248))/36893488147419103232 - sin(q2R)*((1211728953682539*cos(q1R))/2251799813685248 - (3148506117433717*sin(q1R))/4503599627370496)))/42535295865117307932921825928971026432 + (9007199067919185*sin(q3R)*((4774755754024928798560446539205*sin(q2R))/10141204801825835211973625643008 + cos(q2R)*((1211728953682539*cos(q1R))/2251799813685248 - (3148506117433717*sin(q1R))/4503599627370496) + (7514214926474921*sin(q2R)*((3148506117433717*cos(q1R))/4503599627370496 + (1211728953682539*sin(q1R))/2251799813685248))/36893488147419103232))/9007199254740992 + (81129635049124235038645691064225*cos(q3R)*((28359221366286827792295350160645*cos(q1R))/40564819207303340847894502572032 + (10914283902180054573281797610715*sin(q1R))/20282409603651670423947251286016 - 3983318308679801924058395430653/41538374868278621028243970633760768))/81129638414606681695789005144064 - (2115063383689692319117831580025*sin(q3R)*((28359221366286827792295350160645*cos(q1R))/40564819207303340847894502572032 + (10914283902180054573281797610715*sin(q1R))/20282409603651670423947251286016 - 3983318308679801924058395430653/41538374868278621028243970633760768))/10384593717069655257060992658440192 + 46907910686140203564236702804319721336174201386222453025052275/57896044618658097711785492504343953926634992332820282019728792003956564819968))/9007199254740992 + (7514214926474921*sin(q5R)*(((4503599440548691*cos(q4R))/4503599627370496 - (7514214926474921*sin(q4R))/36893488147419103232)*((7514214926474921*sin(q3R)*((4774755754024928798560446539205*cos(q2R))/10141204801825835211973625643008 + (7514214926474921*cos(q2R)*((3148506117433717*cos(q1R))/4503599627370496 + (1211728953682539*sin(q1R))/2251799813685248))/36893488147419103232 - sin(q2R)*((1211728953682539*cos(q1R))/2251799813685248 - (3148506117433717*sin(q1R))/4503599627370496)))/36893488147419103232 - cos(q3R)*((4774755754024928798560446539205*sin(q2R))/10141204801825835211973625643008 + cos(q2R)*((1211728953682539*cos(q1R))/2251799813685248 - (3148506117433717*sin(q1R))/4503599627370496) + (7514214926474921*sin(q2R)*((3148506117433717*cos(q1R))/4503599627370496 + (1211728953682539*sin(q1R))/2251799813685248))/36893488147419103232) + (9007199067919185*sin(q3R)*((28359221366286827792295350160645*cos(q1R))/40564819207303340847894502572032 + (10914283902180054573281797610715*sin(q1R))/20282409603651670423947251286016 - 3983318308679801924058395430653/41538374868278621028243970633760768))/9007199254740992) + ((234819211581865*cos(q4R))/1152921504606846976 + (9007199067919185*sin(q4R))/9007199254740992)*((213097284493758984364555654519459856780913684045*cos(q1R))/1496577676626844588240573268701473812127674924007424 - (43007175577195104036898489188735438973874147925*cos(q2R))/91343852333181432387730302044767688728495783936 + (82012275009546312639155898108543355135168378515*sin(q1R))/748288838313422294120286634350736906063837462003712 - (67682029681889335677290557259385*cos(q2R)*((3148506117433717*cos(q1R))/4503599627370496 + (1211728953682539*sin(q1R))/2251799813685248))/332306998946228968225951765070086144 + (9007199067919185*sin(q2R)*((1211728953682539*cos(q1R))/2251799813685248 - (3148506117433717*sin(q1R))/4503599627370496))/9007199254740992 - 29931509891982604486959633650198707742999153413/1532495540865888858358347027150309183618739122183602176) + (7514214926474921*cos(q4R)*((7514214926474921*cos(q3R)*((4774755754024928798560446539205*cos(q2R))/10141204801825835211973625643008 + (7514214926474921*cos(q2R)*((3148506117433717*cos(q1R))/4503599627370496 + (1211728953682539*sin(q1R))/2251799813685248))/36893488147419103232 - sin(q2R)*((1211728953682539*cos(q1R))/2251799813685248 - (3148506117433717*sin(q1R))/4503599627370496)))/36893488147419103232 + sin(q3R)*((4774755754024928798560446539205*sin(q2R))/10141204801825835211973625643008 + cos(q2R)*((1211728953682539*cos(q1R))/2251799813685248 - (3148506117433717*sin(q1R))/4503599627370496) + (7514214926474921*sin(q2R)*((3148506117433717*cos(q1R))/4503599627370496 + (1211728953682539*sin(q1R))/2251799813685248))/36893488147419103232) + (9007199067919185*cos(q3R)*((28359221366286827792295350160645*cos(q1R))/40564819207303340847894502572032 + (10914283902180054573281797610715*sin(q1R))/20282409603651670423947251286016 - 3983318308679801924058395430653/41538374868278621028243970633760768))/9007199254740992))/36893488147419103232))/36893488147419103232 - cos(q5R)*(((7514214926474921*cos(q4R))/36893488147419103232 + (4503599440548691*sin(q4R))/4503599627370496)*((7514214926474921*sin(q3R)*((4774755754024928798560446539205*cos(q2R))/10141204801825835211973625643008 + (7514214926474921*cos(q2R)*((3148506117433717*cos(q1R))/4503599627370496 + (1211728953682539*sin(q1R))/2251799813685248))/36893488147419103232 - sin(q2R)*((1211728953682539*cos(q1R))/2251799813685248 - (3148506117433717*sin(q1R))/4503599627370496)))/36893488147419103232 - cos(q3R)*((4774755754024928798560446539205*sin(q2R))/10141204801825835211973625643008 + cos(q2R)*((1211728953682539*cos(q1R))/2251799813685248 - (3148506117433717*sin(q1R))/4503599627370496) + (7514214926474921*sin(q2R)*((3148506117433717*cos(q1R))/4503599627370496 + (1211728953682539*sin(q1R))/2251799813685248))/36893488147419103232) + (9007199067919185*sin(q3R)*((28359221366286827792295350160645*cos(q1R))/40564819207303340847894502572032 + (10914283902180054573281797610715*sin(q1R))/20282409603651670423947251286016 - 3983318308679801924058395430653/41538374868278621028243970633760768))/9007199254740992) - ((9007199067919185*cos(q4R))/9007199254740992 - (234819211581865*sin(q4R))/1152921504606846976)*((213097284493758984364555654519459856780913684045*cos(q1R))/1496577676626844588240573268701473812127674924007424 - (43007175577195104036898489188735438973874147925*cos(q2R))/91343852333181432387730302044767688728495783936 + (82012275009546312639155898108543355135168378515*sin(q1R))/748288838313422294120286634350736906063837462003712 - (67682029681889335677290557259385*cos(q2R)*((3148506117433717*cos(q1R))/4503599627370496 + (1211728953682539*sin(q1R))/2251799813685248))/332306998946228968225951765070086144 + (9007199067919185*sin(q2R)*((1211728953682539*cos(q1R))/2251799813685248 - (3148506117433717*sin(q1R))/4503599627370496))/9007199254740992 - 29931509891982604486959633650198707742999153413/1532495540865888858358347027150309183618739122183602176) + (7514214926474921*sin(q4R)*((7514214926474921*cos(q3R)*((4774755754024928798560446539205*cos(q2R))/10141204801825835211973625643008 + (7514214926474921*cos(q2R)*((3148506117433717*cos(q1R))/4503599627370496 + (1211728953682539*sin(q1R))/2251799813685248))/36893488147419103232 - sin(q2R)*((1211728953682539*cos(q1R))/2251799813685248 - (3148506117433717*sin(q1R))/4503599627370496)))/36893488147419103232 + sin(q3R)*((4774755754024928798560446539205*sin(q2R))/10141204801825835211973625643008 + cos(q2R)*((1211728953682539*cos(q1R))/2251799813685248 - (3148506117433717*sin(q1R))/4503599627370496) + (7514214926474921*sin(q2R)*((3148506117433717*cos(q1R))/4503599627370496 + (1211728953682539*sin(q1R))/2251799813685248))/36893488147419103232) + (9007199067919185*cos(q3R)*((28359221366286827792295350160645*cos(q1R))/40564819207303340847894502572032 + (10914283902180054573281797610715*sin(q1R))/20282409603651670423947251286016 - 3983318308679801924058395430653/41538374868278621028243970633760768))/9007199254740992))/36893488147419103232)))/9007199254740992000 - (2436553109258773196144549622003023*sin(q6R)*(sin(q5R)*(((7514214926474921*cos(q4R))/36893488147419103232 + (4503599440548691*sin(q4R))/4503599627370496)*((7514214926474921*sin(q3R)*((4774755754024928798560446539205*cos(q2R))/10141204801825835211973625643008 + (7514214926474921*cos(q2R)*((3148506117433717*cos(q1R))/4503599627370496 + (1211728953682539*sin(q1R))/2251799813685248))/36893488147419103232 - sin(q2R)*((1211728953682539*cos(q1R))/2251799813685248 - (3148506117433717*sin(q1R))/4503599627370496)))/36893488147419103232 - cos(q3R)*((4774755754024928798560446539205*sin(q2R))/10141204801825835211973625643008 + cos(q2R)*((1211728953682539*cos(q1R))/2251799813685248 - (3148506117433717*sin(q1R))/4503599627370496) + (7514214926474921*sin(q2R)*((3148506117433717*cos(q1R))/4503599627370496 + (1211728953682539*sin(q1R))/2251799813685248))/36893488147419103232) + (9007199067919185*sin(q3R)*((28359221366286827792295350160645*cos(q1R))/40564819207303340847894502572032 + (10914283902180054573281797610715*sin(q1R))/20282409603651670423947251286016 - 3983318308679801924058395430653/41538374868278621028243970633760768))/9007199254740992) - ((9007199067919185*cos(q4R))/9007199254740992 - (234819211581865*sin(q4R))/1152921504606846976)*((213097284493758984364555654519459856780913684045*cos(q1R))/1496577676626844588240573268701473812127674924007424 - (43007175577195104036898489188735438973874147925*cos(q2R))/91343852333181432387730302044767688728495783936 + (82012275009546312639155898108543355135168378515*sin(q1R))/748288838313422294120286634350736906063837462003712 - (67682029681889335677290557259385*cos(q2R)*((3148506117433717*cos(q1R))/4503599627370496 + (1211728953682539*sin(q1R))/2251799813685248))/332306998946228968225951765070086144 + (9007199067919185*sin(q2R)*((1211728953682539*cos(q1R))/2251799813685248 - (3148506117433717*sin(q1R))/4503599627370496))/9007199254740992 - 29931509891982604486959633650198707742999153413/1532495540865888858358347027150309183618739122183602176) + (7514214926474921*sin(q4R)*((7514214926474921*cos(q3R)*((4774755754024928798560446539205*cos(q2R))/10141204801825835211973625643008 + (7514214926474921*cos(q2R)*((3148506117433717*cos(q1R))/4503599627370496 + (1211728953682539*sin(q1R))/2251799813685248))/36893488147419103232 - sin(q2R)*((1211728953682539*cos(q1R))/2251799813685248 - (3148506117433717*sin(q1R))/4503599627370496)))/36893488147419103232 + sin(q3R)*((4774755754024928798560446539205*sin(q2R))/10141204801825835211973625643008 + cos(q2R)*((1211728953682539*cos(q1R))/2251799813685248 - (3148506117433717*sin(q1R))/4503599627370496) + (7514214926474921*sin(q2R)*((3148506117433717*cos(q1R))/4503599627370496 + (1211728953682539*sin(q1R))/2251799813685248))/36893488147419103232) + (9007199067919185*cos(q3R)*((28359221366286827792295350160645*cos(q1R))/40564819207303340847894502572032 + (10914283902180054573281797610715*sin(q1R))/20282409603651670423947251286016 - 3983318308679801924058395430653/41538374868278621028243970633760768))/9007199254740992))/36893488147419103232) + (9007199067919185*cos(q5R)*((67399765602155231606998903473897443684277400996768941497011875*cos(q2R))/3450873173395281893717377931138512726225554486085193277581262111899648 - (333960713126929533372903469589741180908441336378844163830032875*cos(q1R))/56539106072908298546665520023773392506479484700019806659891398441363832832 - (128527577967104929471702655059245076724477257328642562920515125*sin(q1R))/28269553036454149273332760011886696253239742350009903329945699220681916416 + (106069577339469832923929692356850887620017617375*cos(q2R)*((3148506117433717*cos(q1R))/4503599627370496 + (1211728953682539*sin(q1R))/2251799813685248))/12554203470773361527671578846415332832204710888928069025792 + (67682029681889335677290557259385*cos(q3R)*((4774755754024928798560446539205*cos(q2R))/10141204801825835211973625643008 + (7514214926474921*cos(q2R)*((3148506117433717*cos(q1R))/4503599627370496 + (1211728953682539*sin(q1R))/2251799813685248))/36893488147419103232 - sin(q2R)*((1211728953682539*cos(q1R))/2251799813685248 - (3148506117433717*sin(q1R))/4503599627370496)))/332306998946228968225951765070086144 - (14115856197532180673579726082375*sin(q2R)*((1211728953682539*cos(q1R))/2251799813685248 - (3148506117433717*sin(q1R))/4503599627370496))/340282366920938463463374607431768211456 + (234819211581865*cos(q3R)*((4774755754024928798560446539205*sin(q2R))/10141204801825835211973625643008 + cos(q2R)*((1211728953682539*cos(q1R))/2251799813685248 - (3148506117433717*sin(q1R))/4503599627370496) + (7514214926474921*sin(q2R)*((3148506117433717*cos(q1R))/4503599627370496 + (1211728953682539*sin(q1R))/2251799813685248))/36893488147419103232))/1152921504606846976 - (1764482024691522628700660907665*sin(q3R)*((4774755754024928798560446539205*cos(q2R))/10141204801825835211973625643008 + (7514214926474921*cos(q2R)*((3148506117433717*cos(q1R))/4503599627370496 + (1211728953682539*sin(q1R))/2251799813685248))/36893488147419103232 - sin(q2R)*((1211728953682539*cos(q1R))/2251799813685248 - (3148506117433717*sin(q1R))/4503599627370496)))/42535295865117307932921825928971026432 + (9007199067919185*sin(q3R)*((4774755754024928798560446539205*sin(q2R))/10141204801825835211973625643008 + cos(q2R)*((1211728953682539*cos(q1R))/2251799813685248 - (3148506117433717*sin(q1R))/4503599627370496) + (7514214926474921*sin(q2R)*((3148506117433717*cos(q1R))/4503599627370496 + (1211728953682539*sin(q1R))/2251799813685248))/36893488147419103232))/9007199254740992 + (81129635049124235038645691064225*cos(q3R)*((28359221366286827792295350160645*cos(q1R))/40564819207303340847894502572032 + (10914283902180054573281797610715*sin(q1R))/20282409603651670423947251286016 - 3983318308679801924058395430653/41538374868278621028243970633760768))/81129638414606681695789005144064 - (2115063383689692319117831580025*sin(q3R)*((28359221366286827792295350160645*cos(q1R))/40564819207303340847894502572032 + (10914283902180054573281797610715*sin(q1R))/20282409603651670423947251286016 - 3983318308679801924058395430653/41538374868278621028243970633760768))/10384593717069655257060992658440192 + 46907910686140203564236702804319721336174201386222453025052275/57896044618658097711785492504343953926634992332820282019728792003956564819968))/9007199254740992 + (7514214926474921*cos(q5R)*(((4503599440548691*cos(q4R))/4503599627370496 - (7514214926474921*sin(q4R))/36893488147419103232)*((7514214926474921*sin(q3R)*((4774755754024928798560446539205*cos(q2R))/10141204801825835211973625643008 + (7514214926474921*cos(q2R)*((3148506117433717*cos(q1R))/4503599627370496 + (1211728953682539*sin(q1R))/2251799813685248))/36893488147419103232 - sin(q2R)*((1211728953682539*cos(q1R))/2251799813685248 - (3148506117433717*sin(q1R))/4503599627370496)))/36893488147419103232 - cos(q3R)*((4774755754024928798560446539205*sin(q2R))/10141204801825835211973625643008 + cos(q2R)*((1211728953682539*cos(q1R))/2251799813685248 - (3148506117433717*sin(q1R))/4503599627370496) + (7514214926474921*sin(q2R)*((3148506117433717*cos(q1R))/4503599627370496 + (1211728953682539*sin(q1R))/2251799813685248))/36893488147419103232) + (9007199067919185*sin(q3R)*((28359221366286827792295350160645*cos(q1R))/40564819207303340847894502572032 + (10914283902180054573281797610715*sin(q1R))/20282409603651670423947251286016 - 3983318308679801924058395430653/41538374868278621028243970633760768))/9007199254740992) + ((234819211581865*cos(q4R))/1152921504606846976 + (9007199067919185*sin(q4R))/9007199254740992)*((213097284493758984364555654519459856780913684045*cos(q1R))/1496577676626844588240573268701473812127674924007424 - (43007175577195104036898489188735438973874147925*cos(q2R))/91343852333181432387730302044767688728495783936 + (82012275009546312639155898108543355135168378515*sin(q1R))/748288838313422294120286634350736906063837462003712 - (67682029681889335677290557259385*cos(q2R)*((3148506117433717*cos(q1R))/4503599627370496 + (1211728953682539*sin(q1R))/2251799813685248))/332306998946228968225951765070086144 + (9007199067919185*sin(q2R)*((1211728953682539*cos(q1R))/2251799813685248 - (3148506117433717*sin(q1R))/4503599627370496))/9007199254740992 - 29931509891982604486959633650198707742999153413/1532495540865888858358347027150309183618739122183602176) + (7514214926474921*cos(q4R)*((7514214926474921*cos(q3R)*((4774755754024928798560446539205*cos(q2R))/10141204801825835211973625643008 + (7514214926474921*cos(q2R)*((3148506117433717*cos(q1R))/4503599627370496 + (1211728953682539*sin(q1R))/2251799813685248))/36893488147419103232 - sin(q2R)*((1211728953682539*cos(q1R))/2251799813685248 - (3148506117433717*sin(q1R))/4503599627370496)))/36893488147419103232 + sin(q3R)*((4774755754024928798560446539205*sin(q2R))/10141204801825835211973625643008 + cos(q2R)*((1211728953682539*cos(q1R))/2251799813685248 - (3148506117433717*sin(q1R))/4503599627370496) + (7514214926474921*sin(q2R)*((3148506117433717*cos(q1R))/4503599627370496 + (1211728953682539*sin(q1R))/2251799813685248))/36893488147419103232) + (9007199067919185*cos(q3R)*((28359221366286827792295350160645*cos(q1R))/40564819207303340847894502572032 + (10914283902180054573281797610715*sin(q1R))/20282409603651670423947251286016 - 3983318308679801924058395430653/41538374868278621028243970633760768))/9007199254740992))/36893488147419103232))/36893488147419103232))/332306998946228968225951765070086144000 + (27*sin(q6R)*((9007199067919185*sin(q5R)*((67399765602155231606998903473897443684277400996768941497011875*cos(q2R))/3450873173395281893717377931138512726225554486085193277581262111899648 - (333960713126929533372903469589741180908441336378844163830032875*cos(q1R))/56539106072908298546665520023773392506479484700019806659891398441363832832 - (128527577967104929471702655059245076724477257328642562920515125*sin(q1R))/28269553036454149273332760011886696253239742350009903329945699220681916416 + (106069577339469832923929692356850887620017617375*cos(q2R)*((3148506117433717*cos(q1R))/4503599627370496 + (1211728953682539*sin(q1R))/2251799813685248))/12554203470773361527671578846415332832204710888928069025792 + (67682029681889335677290557259385*cos(q3R)*((4774755754024928798560446539205*cos(q2R))/10141204801825835211973625643008 + (7514214926474921*cos(q2R)*((3148506117433717*cos(q1R))/4503599627370496 + (1211728953682539*sin(q1R))/2251799813685248))/36893488147419103232 - sin(q2R)*((1211728953682539*cos(q1R))/2251799813685248 - (3148506117433717*sin(q1R))/4503599627370496)))/332306998946228968225951765070086144 - (14115856197532180673579726082375*sin(q2R)*((1211728953682539*cos(q1R))/2251799813685248 - (3148506117433717*sin(q1R))/4503599627370496))/340282366920938463463374607431768211456 + (234819211581865*cos(q3R)*((4774755754024928798560446539205*sin(q2R))/10141204801825835211973625643008 + cos(q2R)*((1211728953682539*cos(q1R))/2251799813685248 - (3148506117433717*sin(q1R))/4503599627370496) + (7514214926474921*sin(q2R)*((3148506117433717*cos(q1R))/4503599627370496 + (1211728953682539*sin(q1R))/2251799813685248))/36893488147419103232))/1152921504606846976 - (1764482024691522628700660907665*sin(q3R)*((4774755754024928798560446539205*cos(q2R))/10141204801825835211973625643008 + (7514214926474921*cos(q2R)*((3148506117433717*cos(q1R))/4503599627370496 + (1211728953682539*sin(q1R))/2251799813685248))/36893488147419103232 - sin(q2R)*((1211728953682539*cos(q1R))/2251799813685248 - (3148506117433717*sin(q1R))/4503599627370496)))/42535295865117307932921825928971026432 + (9007199067919185*sin(q3R)*((4774755754024928798560446539205*sin(q2R))/10141204801825835211973625643008 + cos(q2R)*((1211728953682539*cos(q1R))/2251799813685248 - (3148506117433717*sin(q1R))/4503599627370496) + (7514214926474921*sin(q2R)*((3148506117433717*cos(q1R))/4503599627370496 + (1211728953682539*sin(q1R))/2251799813685248))/36893488147419103232))/9007199254740992 + (81129635049124235038645691064225*cos(q3R)*((28359221366286827792295350160645*cos(q1R))/40564819207303340847894502572032 + (10914283902180054573281797610715*sin(q1R))/20282409603651670423947251286016 - 3983318308679801924058395430653/41538374868278621028243970633760768))/81129638414606681695789005144064 - (2115063383689692319117831580025*sin(q3R)*((28359221366286827792295350160645*cos(q1R))/40564819207303340847894502572032 + (10914283902180054573281797610715*sin(q1R))/20282409603651670423947251286016 - 3983318308679801924058395430653/41538374868278621028243970633760768))/10384593717069655257060992658440192 + 46907910686140203564236702804319721336174201386222453025052275/57896044618658097711785492504343953926634992332820282019728792003956564819968))/9007199254740992 + (7514214926474921*sin(q5R)*(((4503599440548691*cos(q4R))/4503599627370496 - (7514214926474921*sin(q4R))/36893488147419103232)*((7514214926474921*sin(q3R)*((4774755754024928798560446539205*cos(q2R))/10141204801825835211973625643008 + (7514214926474921*cos(q2R)*((3148506117433717*cos(q1R))/4503599627370496 + (1211728953682539*sin(q1R))/2251799813685248))/36893488147419103232 - sin(q2R)*((1211728953682539*cos(q1R))/2251799813685248 - (3148506117433717*sin(q1R))/4503599627370496)))/36893488147419103232 - cos(q3R)*((4774755754024928798560446539205*sin(q2R))/10141204801825835211973625643008 + cos(q2R)*((1211728953682539*cos(q1R))/2251799813685248 - (3148506117433717*sin(q1R))/4503599627370496) + (7514214926474921*sin(q2R)*((3148506117433717*cos(q1R))/4503599627370496 + (1211728953682539*sin(q1R))/2251799813685248))/36893488147419103232) + (9007199067919185*sin(q3R)*((28359221366286827792295350160645*cos(q1R))/40564819207303340847894502572032 + (10914283902180054573281797610715*sin(q1R))/20282409603651670423947251286016 - 3983318308679801924058395430653/41538374868278621028243970633760768))/9007199254740992) + ((234819211581865*cos(q4R))/1152921504606846976 + (9007199067919185*sin(q4R))/9007199254740992)*((213097284493758984364555654519459856780913684045*cos(q1R))/1496577676626844588240573268701473812127674924007424 - (43007175577195104036898489188735438973874147925*cos(q2R))/91343852333181432387730302044767688728495783936 + (82012275009546312639155898108543355135168378515*sin(q1R))/748288838313422294120286634350736906063837462003712 - (67682029681889335677290557259385*cos(q2R)*((3148506117433717*cos(q1R))/4503599627370496 + (1211728953682539*sin(q1R))/2251799813685248))/332306998946228968225951765070086144 + (9007199067919185*sin(q2R)*((1211728953682539*cos(q1R))/2251799813685248 - (3148506117433717*sin(q1R))/4503599627370496))/9007199254740992 - 29931509891982604486959633650198707742999153413/1532495540865888858358347027150309183618739122183602176) + (7514214926474921*cos(q4R)*((7514214926474921*cos(q3R)*((4774755754024928798560446539205*cos(q2R))/10141204801825835211973625643008 + (7514214926474921*cos(q2R)*((3148506117433717*cos(q1R))/4503599627370496 + (1211728953682539*sin(q1R))/2251799813685248))/36893488147419103232 - sin(q2R)*((1211728953682539*cos(q1R))/2251799813685248 - (3148506117433717*sin(q1R))/4503599627370496)))/36893488147419103232 + sin(q3R)*((4774755754024928798560446539205*sin(q2R))/10141204801825835211973625643008 + cos(q2R)*((1211728953682539*cos(q1R))/2251799813685248 - (3148506117433717*sin(q1R))/4503599627370496) + (7514214926474921*sin(q2R)*((3148506117433717*cos(q1R))/4503599627370496 + (1211728953682539*sin(q1R))/2251799813685248))/36893488147419103232) + (9007199067919185*cos(q3R)*((28359221366286827792295350160645*cos(q1R))/40564819207303340847894502572032 + (10914283902180054573281797610715*sin(q1R))/20282409603651670423947251286016 - 3983318308679801924058395430653/41538374868278621028243970633760768))/9007199254740992))/36893488147419103232))/36893488147419103232 - cos(q5R)*(((7514214926474921*cos(q4R))/36893488147419103232 + (4503599440548691*sin(q4R))/4503599627370496)*((7514214926474921*sin(q3R)*((4774755754024928798560446539205*cos(q2R))/10141204801825835211973625643008 + (7514214926474921*cos(q2R)*((3148506117433717*cos(q1R))/4503599627370496 + (1211728953682539*sin(q1R))/2251799813685248))/36893488147419103232 - sin(q2R)*((1211728953682539*cos(q1R))/2251799813685248 - (3148506117433717*sin(q1R))/4503599627370496)))/36893488147419103232 - cos(q3R)*((4774755754024928798560446539205*sin(q2R))/10141204801825835211973625643008 + cos(q2R)*((1211728953682539*cos(q1R))/2251799813685248 - (3148506117433717*sin(q1R))/4503599627370496) + (7514214926474921*sin(q2R)*((3148506117433717*cos(q1R))/4503599627370496 + (1211728953682539*sin(q1R))/2251799813685248))/36893488147419103232) + (9007199067919185*sin(q3R)*((28359221366286827792295350160645*cos(q1R))/40564819207303340847894502572032 + (10914283902180054573281797610715*sin(q1R))/20282409603651670423947251286016 - 3983318308679801924058395430653/41538374868278621028243970633760768))/9007199254740992) - ((9007199067919185*cos(q4R))/9007199254740992 - (234819211581865*sin(q4R))/1152921504606846976)*((213097284493758984364555654519459856780913684045*cos(q1R))/1496577676626844588240573268701473812127674924007424 - (43007175577195104036898489188735438973874147925*cos(q2R))/91343852333181432387730302044767688728495783936 + (82012275009546312639155898108543355135168378515*sin(q1R))/748288838313422294120286634350736906063837462003712 - (67682029681889335677290557259385*cos(q2R)*((3148506117433717*cos(q1R))/4503599627370496 + (1211728953682539*sin(q1R))/2251799813685248))/332306998946228968225951765070086144 + (9007199067919185*sin(q2R)*((1211728953682539*cos(q1R))/2251799813685248 - (3148506117433717*sin(q1R))/4503599627370496))/9007199254740992 - 29931509891982604486959633650198707742999153413/1532495540865888858358347027150309183618739122183602176) + (7514214926474921*sin(q4R)*((7514214926474921*cos(q3R)*((4774755754024928798560446539205*cos(q2R))/10141204801825835211973625643008 + (7514214926474921*cos(q2R)*((3148506117433717*cos(q1R))/4503599627370496 + (1211728953682539*sin(q1R))/2251799813685248))/36893488147419103232 - sin(q2R)*((1211728953682539*cos(q1R))/2251799813685248 - (3148506117433717*sin(q1R))/4503599627370496)))/36893488147419103232 + sin(q3R)*((4774755754024928798560446539205*sin(q2R))/10141204801825835211973625643008 + cos(q2R)*((1211728953682539*cos(q1R))/2251799813685248 - (3148506117433717*sin(q1R))/4503599627370496) + (7514214926474921*sin(q2R)*((3148506117433717*cos(q1R))/4503599627370496 + (1211728953682539*sin(q1R))/2251799813685248))/36893488147419103232) + (9007199067919185*cos(q3R)*((28359221366286827792295350160645*cos(q1R))/40564819207303340847894502572032 + (10914283902180054573281797610715*sin(q1R))/20282409603651670423947251286016 - 3983318308679801924058395430653/41538374868278621028243970633760768))/9007199254740992))/36893488147419103232)))/1000 + (48638874966763599*cos(q6R)*((2509452575434582988059840876067412966740105600591515474393999405526015293027875*cos(q1R))/2085924839766513752338888384931203236916703635113918720651407820138886450957656787131798913024 - (506456324728625783189839291299220948962368525946389165528853917988948626686875*cos(q2R))/127314748520905380391777855525586135065716774604121015664758778084648831235208544136462336 + (965783844824089043900160825489639266458473927649494297144005158508529713680125*sin(q1R))/1042962419883256876169444192465601618458351817556959360325703910069443225478828393565899456512 - (797029601289130257223357069404502671534492977261568326111352375*cos(q2R)*((3148506117433717*cos(q1R))/4503599627370496 + (1211728953682539*sin(q1R))/2251799813685248))/463168356949264781694283940034751631413079938662562256157830336031652518559744 - (508577317689771495245073589786522929324694383585*cos(q3R)*((4774755754024928798560446539205*cos(q2R))/10141204801825835211973625643008 + (7514214926474921*cos(q2R)*((3148506117433717*cos(q1R))/4503599627370496 + (1211728953682539*sin(q1R))/2251799813685248))/36893488147419103232 - sin(q2R)*((1211728953682539*cos(q1R))/2251799813685248 - (3148506117433717*sin(q1R))/4503599627370496)))/12259964326927110866866776217202473468949912977468817408 + (9007199067919185*((4503599440548691*cos(q4R))/4503599627370496 - (7514214926474921*sin(q4R))/36893488147419103232)*((7514214926474921*sin(q3R)*((4774755754024928798560446539205*cos(q2R))/10141204801825835211973625643008 + (7514214926474921*cos(q2R)*((3148506117433717*cos(q1R))/4503599627370496 + (1211728953682539*sin(q1R))/2251799813685248))/36893488147419103232 - sin(q2R)*((1211728953682539*cos(q1R))/2251799813685248 - (3148506117433717*sin(q1R))/4503599627370496)))/36893488147419103232 - cos(q3R)*((4774755754024928798560446539205*sin(q2R))/10141204801825835211973625643008 + cos(q2R)*((1211728953682539*cos(q1R))/2251799813685248 - (3148506117433717*sin(q1R))/4503599627370496) + (7514214926474921*sin(q2R)*((3148506117433717*cos(q1R))/4503599627370496 + (1211728953682539*sin(q1R))/2251799813685248))/36893488147419103232) + (9007199067919185*sin(q3R)*((28359221366286827792295350160645*cos(q1R))/40564819207303340847894502572032 + (10914283902180054573281797610715*sin(q1R))/20282409603651670423947251286016 - 3983318308679801924058395430653/41538374868278621028243970633760768))/9007199254740992))/9007199254740992 + (106069577339469832923929692356850887620017617375*sin(q2R)*((1211728953682539*cos(q1R))/2251799813685248 - (3148506117433717*sin(q1R))/4503599627370496))/12554203470773361527671578846415332832204710888928069025792 - (1764482024691522628700660907665*cos(q3R)*((4774755754024928798560446539205*sin(q2R))/10141204801825835211973625643008 + cos(q2R)*((1211728953682539*cos(q1R))/2251799813685248 - (3148506117433717*sin(q1R))/4503599627370496) + (7514214926474921*sin(q2R)*((3148506117433717*cos(q1R))/4503599627370496 + (1211728953682539*sin(q1R))/2251799813685248))/36893488147419103232))/42535295865117307932921825928971026432 + (13258697167433729449897784796786197386719169465*sin(q3R)*((4774755754024928798560446539205*cos(q2R))/10141204801825835211973625643008 + (7514214926474921*cos(q2R)*((3148506117433717*cos(q1R))/4503599627370496 + (1211728953682539*sin(q1R))/2251799813685248))/36893488147419103232 - sin(q2R)*((1211728953682539*cos(q1R))/2251799813685248 - (3148506117433717*sin(q1R))/4503599627370496)))/1569275433846670190958947355801916604025588861116008628224 + (9007199067919185*((234819211581865*cos(q4R))/1152921504606846976 + (9007199067919185*sin(q4R))/9007199254740992)*((213097284493758984364555654519459856780913684045*cos(q1R))/1496577676626844588240573268701473812127674924007424 - (43007175577195104036898489188735438973874147925*cos(q2R))/91343852333181432387730302044767688728495783936 + (82012275009546312639155898108543355135168378515*sin(q1R))/748288838313422294120286634350736906063837462003712 - (67682029681889335677290557259385*cos(q2R)*((3148506117433717*cos(q1R))/4503599627370496 + (1211728953682539*sin(q1R))/2251799813685248))/332306998946228968225951765070086144 + (9007199067919185*sin(q2R)*((1211728953682539*cos(q1R))/2251799813685248 - (3148506117433717*sin(q1R))/4503599627370496))/9007199254740992 - 29931509891982604486959633650198707742999153413/1532495540865888858358347027150309183618739122183602176))/9007199254740992 - (67682029681889335677290557259385*sin(q3R)*((4774755754024928798560446539205*sin(q2R))/10141204801825835211973625643008 + cos(q2R)*((1211728953682539*cos(q1R))/2251799813685248 - (3148506117433717*sin(q1R))/4503599627370496) + (7514214926474921*sin(q2R)*((3148506117433717*cos(q1R))/4503599627370496 + (1211728953682539*sin(q1R))/2251799813685248))/36893488147419103232))/332306998946228968225951765070086144 + (67682029681889335677290557259385*cos(q4R)*((7514214926474921*cos(q3R)*((4774755754024928798560446539205*cos(q2R))/10141204801825835211973625643008 + (7514214926474921*cos(q2R)*((3148506117433717*cos(q1R))/4503599627370496 + (1211728953682539*sin(q1R))/2251799813685248))/36893488147419103232 - sin(q2R)*((1211728953682539*cos(q1R))/2251799813685248 - (3148506117433717*sin(q1R))/4503599627370496)))/36893488147419103232 + sin(q3R)*((4774755754024928798560446539205*sin(q2R))/10141204801825835211973625643008 + cos(q2R)*((1211728953682539*cos(q1R))/2251799813685248 - (3148506117433717*sin(q1R))/4503599627370496) + (7514214926474921*sin(q2R)*((3148506117433717*cos(q1R))/4503599627370496 + (1211728953682539*sin(q1R))/2251799813685248))/36893488147419103232) + (9007199067919185*cos(q3R)*((28359221366286827792295350160645*cos(q1R))/40564819207303340847894502572032 + (10914283902180054573281797610715*sin(q1R))/20282409603651670423947251286016 - 3983318308679801924058395430653/41538374868278621028243970633760768))/9007199254740992))/332306998946228968225951765070086144 - (609625514665592237562888769449172969868262801225*cos(q3R)*((28359221366286827792295350160645*cos(q1R))/40564819207303340847894502572032 + (10914283902180054573281797610715*sin(q1R))/20282409603651670423947251286016 - 3983318308679801924058395430653/41538374868278621028243970633760768))/2993155353253689176481146537402947624255349848014848 + (15893040848161638993908057577265778144967053025*sin(q3R)*((28359221366286827792295350160645*cos(q1R))/40564819207303340847894502572032 + (10914283902180054573281797610715*sin(q1R))/20282409603651670423947251286016 - 3983318308679801924058395430653/41538374868278621028243970633760768))/383123885216472214589586756787577295904684780545900544 - 352476122647547170802038223626176166472971174169179835173727810348367501495275/2135987035920910082395021706169552114602704522356652769947041607822219725780640550022962086936576))/1801439850948198400 - (584133382113593486367040631332731*sin(q6R)*((2509452575434582988059840876067412966740105600591515474393999405526015293027875*cos(q1R))/2085924839766513752338888384931203236916703635113918720651407820138886450957656787131798913024 - (506456324728625783189839291299220948962368525946389165528853917988948626686875*cos(q2R))/127314748520905380391777855525586135065716774604121015664758778084648831235208544136462336 + (965783844824089043900160825489639266458473927649494297144005158508529713680125*sin(q1R))/1042962419883256876169444192465601618458351817556959360325703910069443225478828393565899456512 - (797029601289130257223357069404502671534492977261568326111352375*cos(q2R)*((3148506117433717*cos(q1R))/4503599627370496 + (1211728953682539*sin(q1R))/2251799813685248))/463168356949264781694283940034751631413079938662562256157830336031652518559744 - (508577317689771495245073589786522929324694383585*cos(q3R)*((4774755754024928798560446539205*cos(q2R))/10141204801825835211973625643008 + (7514214926474921*cos(q2R)*((3148506117433717*cos(q1R))/4503599627370496 + (1211728953682539*sin(q1R))/2251799813685248))/36893488147419103232 - sin(q2R)*((1211728953682539*cos(q1R))/2251799813685248 - (3148506117433717*sin(q1R))/4503599627370496)))/12259964326927110866866776217202473468949912977468817408 + (9007199067919185*((4503599440548691*cos(q4R))/4503599627370496 - (7514214926474921*sin(q4R))/36893488147419103232)*((7514214926474921*sin(q3R)*((4774755754024928798560446539205*cos(q2R))/10141204801825835211973625643008 + (7514214926474921*cos(q2R)*((3148506117433717*cos(q1R))/4503599627370496 + (1211728953682539*sin(q1R))/2251799813685248))/36893488147419103232 - sin(q2R)*((1211728953682539*cos(q1R))/2251799813685248 - (3148506117433717*sin(q1R))/4503599627370496)))/36893488147419103232 - cos(q3R)*((4774755754024928798560446539205*sin(q2R))/10141204801825835211973625643008 + cos(q2R)*((1211728953682539*cos(q1R))/2251799813685248 - (3148506117433717*sin(q1R))/4503599627370496) + (7514214926474921*sin(q2R)*((3148506117433717*cos(q1R))/4503599627370496 + (1211728953682539*sin(q1R))/2251799813685248))/36893488147419103232) + (9007199067919185*sin(q3R)*((28359221366286827792295350160645*cos(q1R))/40564819207303340847894502572032 + (10914283902180054573281797610715*sin(q1R))/20282409603651670423947251286016 - 3983318308679801924058395430653/41538374868278621028243970633760768))/9007199254740992))/9007199254740992 + (106069577339469832923929692356850887620017617375*sin(q2R)*((1211728953682539*cos(q1R))/2251799813685248 - (3148506117433717*sin(q1R))/4503599627370496))/12554203470773361527671578846415332832204710888928069025792 - (1764482024691522628700660907665*cos(q3R)*((4774755754024928798560446539205*sin(q2R))/10141204801825835211973625643008 + cos(q2R)*((1211728953682539*cos(q1R))/2251799813685248 - (3148506117433717*sin(q1R))/4503599627370496) + (7514214926474921*sin(q2R)*((3148506117433717*cos(q1R))/4503599627370496 + (1211728953682539*sin(q1R))/2251799813685248))/36893488147419103232))/42535295865117307932921825928971026432 + (13258697167433729449897784796786197386719169465*sin(q3R)*((4774755754024928798560446539205*cos(q2R))/10141204801825835211973625643008 + (7514214926474921*cos(q2R)*((3148506117433717*cos(q1R))/4503599627370496 + (1211728953682539*sin(q1R))/2251799813685248))/36893488147419103232 - sin(q2R)*((1211728953682539*cos(q1R))/2251799813685248 - (3148506117433717*sin(q1R))/4503599627370496)))/1569275433846670190958947355801916604025588861116008628224 + (9007199067919185*((234819211581865*cos(q4R))/1152921504606846976 + (9007199067919185*sin(q4R))/9007199254740992)*((213097284493758984364555654519459856780913684045*cos(q1R))/1496577676626844588240573268701473812127674924007424 - (43007175577195104036898489188735438973874147925*cos(q2R))/91343852333181432387730302044767688728495783936 + (82012275009546312639155898108543355135168378515*sin(q1R))/748288838313422294120286634350736906063837462003712 - (67682029681889335677290557259385*cos(q2R)*((3148506117433717*cos(q1R))/4503599627370496 + (1211728953682539*sin(q1R))/2251799813685248))/332306998946228968225951765070086144 + (9007199067919185*sin(q2R)*((1211728953682539*cos(q1R))/2251799813685248 - (3148506117433717*sin(q1R))/4503599627370496))/9007199254740992 - 29931509891982604486959633650198707742999153413/1532495540865888858358347027150309183618739122183602176))/9007199254740992 - (67682029681889335677290557259385*sin(q3R)*((4774755754024928798560446539205*sin(q2R))/10141204801825835211973625643008 + cos(q2R)*((1211728953682539*cos(q1R))/2251799813685248 - (3148506117433717*sin(q1R))/4503599627370496) + (7514214926474921*sin(q2R)*((3148506117433717*cos(q1R))/4503599627370496 + (1211728953682539*sin(q1R))/2251799813685248))/36893488147419103232))/332306998946228968225951765070086144 + (67682029681889335677290557259385*cos(q4R)*((7514214926474921*cos(q3R)*((4774755754024928798560446539205*cos(q2R))/10141204801825835211973625643008 + (7514214926474921*cos(q2R)*((3148506117433717*cos(q1R))/4503599627370496 + (1211728953682539*sin(q1R))/2251799813685248))/36893488147419103232 - sin(q2R)*((1211728953682539*cos(q1R))/2251799813685248 - (3148506117433717*sin(q1R))/4503599627370496)))/36893488147419103232 + sin(q3R)*((4774755754024928798560446539205*sin(q2R))/10141204801825835211973625643008 + cos(q2R)*((1211728953682539*cos(q1R))/2251799813685248 - (3148506117433717*sin(q1R))/4503599627370496) + (7514214926474921*sin(q2R)*((3148506117433717*cos(q1R))/4503599627370496 + (1211728953682539*sin(q1R))/2251799813685248))/36893488147419103232) + (9007199067919185*cos(q3R)*((28359221366286827792295350160645*cos(q1R))/40564819207303340847894502572032 + (10914283902180054573281797610715*sin(q1R))/20282409603651670423947251286016 - 3983318308679801924058395430653/41538374868278621028243970633760768))/9007199254740992))/332306998946228968225951765070086144 - (609625514665592237562888769449172969868262801225*cos(q3R)*((28359221366286827792295350160645*cos(q1R))/40564819207303340847894502572032 + (10914283902180054573281797610715*sin(q1R))/20282409603651670423947251286016 - 3983318308679801924058395430653/41538374868278621028243970633760768))/2993155353253689176481146537402947624255349848014848 + (15893040848161638993908057577265778144967053025*sin(q3R)*((28359221366286827792295350160645*cos(q1R))/40564819207303340847894502572032 + (10914283902180054573281797610715*sin(q1R))/20282409603651670423947251286016 - 3983318308679801924058395430653/41538374868278621028243970633760768))/383123885216472214589586756787577295904684780545900544 - 352476122647547170802038223626176166472971174169179835173727810348367501495275/2135987035920910082395021706169552114602704522356652769947041607822219725780640550022962086936576))/16225927682921336339157801028812800 + (202883803014822867*cos(q6R)*(sin(q5R)*(((7514214926474921*cos(q4R))/36893488147419103232 + (4503599440548691*sin(q4R))/4503599627370496)*((7514214926474921*sin(q3R)*((4774755754024928798560446539205*cos(q2R))/10141204801825835211973625643008 + (7514214926474921*cos(q2R)*((3148506117433717*cos(q1R))/4503599627370496 + (1211728953682539*sin(q1R))/2251799813685248))/36893488147419103232 - sin(q2R)*((1211728953682539*cos(q1R))/2251799813685248 - (3148506117433717*sin(q1R))/4503599627370496)))/36893488147419103232 - cos(q3R)*((4774755754024928798560446539205*sin(q2R))/10141204801825835211973625643008 + cos(q2R)*((1211728953682539*cos(q1R))/2251799813685248 - (3148506117433717*sin(q1R))/4503599627370496) + (7514214926474921*sin(q2R)*((3148506117433717*cos(q1R))/4503599627370496 + (1211728953682539*sin(q1R))/2251799813685248))/36893488147419103232) + (9007199067919185*sin(q3R)*((28359221366286827792295350160645*cos(q1R))/40564819207303340847894502572032 + (10914283902180054573281797610715*sin(q1R))/20282409603651670423947251286016 - 3983318308679801924058395430653/41538374868278621028243970633760768))/9007199254740992) - ((9007199067919185*cos(q4R))/9007199254740992 - (234819211581865*sin(q4R))/1152921504606846976)*((213097284493758984364555654519459856780913684045*cos(q1R))/1496577676626844588240573268701473812127674924007424 - (43007175577195104036898489188735438973874147925*cos(q2R))/91343852333181432387730302044767688728495783936 + (82012275009546312639155898108543355135168378515*sin(q1R))/748288838313422294120286634350736906063837462003712 - (67682029681889335677290557259385*cos(q2R)*((3148506117433717*cos(q1R))/4503599627370496 + (1211728953682539*sin(q1R))/2251799813685248))/332306998946228968225951765070086144 + (9007199067919185*sin(q2R)*((1211728953682539*cos(q1R))/2251799813685248 - (3148506117433717*sin(q1R))/4503599627370496))/9007199254740992 - 29931509891982604486959633650198707742999153413/1532495540865888858358347027150309183618739122183602176) + (7514214926474921*sin(q4R)*((7514214926474921*cos(q3R)*((4774755754024928798560446539205*cos(q2R))/10141204801825835211973625643008 + 